simulink model "TwoLinkCartesianNN"  (Simulink 7.6)
settings: Solver=ode45  StartTime=0.0  StopTime=10.0  RelTol=1e-3
libraries: neural x148, roblocks x3, simulink x1
(part 4 of 5)

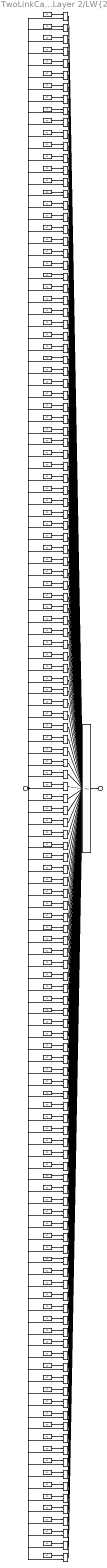
== system TwoLinkCartesianNN/Custom Neural Network/Layer 2/LW{2,1} ==
  "ad{2,1}" : Inport  PortDimensions=10
      mask Display: e = 0.06;c1 = [120 230 180]/255;c2 = ([120 230 180]+0)/(256+128);c3 = ([120 230 180]+128)/(256+128);patch([0 1 1 0],[0 0 1 1],c1);patch([0 1 1 1-e 1-e 0+e],[0 0 1 1-e 0+e 0+e],c2);patch([0 0 1 1-e 0+e 0+e],[0 1 1 1-e 1-e 0+e],c3);plot([0 1 1 0 0],[0 0 1 1 0]);
  "IW{2,1}(1,:)'" : Constant  Value=[1.3771051605919495397500895705888979136943817138671875;1.4379727812980205303716729758889414370059967041015625;-0.71484904480061584042260847127181477844715118408203125;0.195728691276192190429128459072671830654144287109375;-1.40204187084294051857114027370698750019073486328125;-0.0711414545212695481612996672993176616728305816650390625;-0.77472100986854341986287408872158266603946685791015625;1.489410727801894207544819437316618859767913818359375;1.715302916655259135580990914604626595973968505859375;2.718694540405024451246163152973167598247528076171875]
      mask Display: e = 0.06;c1 = [120 150 230]/255;c2 = ([120 150 230]+0)/383;c3 = ([120 150 230]+128)/383;patch([0 1 1 0],[0 0 1 1],c1);patch([0 1 1 1-e 1-e 0+e],[0 0 1 1-e 0+e 0+e],c2);patch([0 0 1 1-e 0+e 0+e],[0 1 1 1-e 1-e 0+e],c3);plot([0 1 1 0 0],[0 0 1 1 0]);disp('weights');
  "IW{2,1}(10,:)'" : Constant  Value=[-1.049488522602133766525867031305097043514251708984375;1.16658805918520958044837243505753576755523681640625;-0.79840961629492712692268696628161706030368804931640625;-0.596367663897474198364534458960406482219696044921875;1.558993573274443544818268492235802114009857177734375;-0.5828639335874774562995526139275170862674713134765625;2.034904616688063327956115244887769222259521484375;-0.74732958615957112424865727007272653281688690185546875;1.8705078039982783177919145600753836333751678466796875;0.39898729108689867661752259664353914558887481689453125]
      mask Display: e = 0.06;c1 = [120 150 230]/255;c2 = ([120 150 230]+0)/383;c3 = ([120 150 230]+128)/383;patch([0 1 1 0],[0 0 1 1],c1);patch([0 1 1 1-e 1-e 0+e],[0 0 1 1-e 0+e 0+e],c2);patch([0 0 1 1-e 0+e 0+e],[0 1 1 1-e 1-e 0+e],c3);plot([0 1 1 0 0],[0 0 1 1 0]);disp('weights');
  "IW{2,1}(100,:)'" : Constant  Value=[-1.225944562580657315464804923976771533489227294921875;0.8399160095312352414254064569831825792789459228515625;0.4059314815768413353680443833582103252410888671875;2.245993199122457983918366153375245630741119384765625;-1.34935754592711010246830483083613216876983642578125;0.88606781850175642123446095865801908075809478759765625;-0.49755438593116918521985780898830853402614593505859375;-2.13120059899219693733130043256096541881561279296875;0.70410764783046941861499590231687761843204498291015625;0.51899870794404001639321677430416457355022430419921875]
      mask Display: e = 0.06;c1 = [120 150 230]/255;c2 = ([120 150 230]+0)/383;c3 = ([120 150 230]+128)/383;patch([0 1 1 0],[0 0 1 1],c1);patch([0 1 1 1-e 1-e 0+e],[0 0 1 1-e 0+e 0+e],c2);patch([0 0 1 1-e 0+e 0+e],[0 1 1 1-e 1-e 0+e],c3);plot([0 1 1 0 0],[0 0 1 1 0]);disp('weights');
  "IW{2,1}(101,:)'" : Constant  Value=[-0.1714405387687350235115246732675586827099323272705078125;-1.843339039992688999092251833644695580005645751953125;0.7673938264733717318222261383198201656341552734375;0.28768398362630309694765173844643868505954742431640625;-1.064859588474557750004123590770177543163299560546875;1.0058133839706095979948941021575592458248138427734375;0.49729546415479652932134513321216218173503875732421875;0.7812040402926265780791936776950024068355560302734375;-1.448282334202080079421648406423628330230712890625;-1.604786002596785277063418106990866363048553466796875]
      mask Display: e = 0.06;c1 = [120 150 230]/255;c2 = ([120 150 230]+0)/383;c3 = ([120 150 230]+128)/383;patch([0 1 1 0],[0 0 1 1],c1);patch([0 1 1 1-e 1-e 0+e],[0 0 1 1-e 0+e 0+e],c2);patch([0 0 1 1-e 0+e 0+e],[0 1 1 1-e 1-e 0+e],c3);plot([0 1 1 0 0],[0 0 1 1 0]);disp('weights');
  "IW{2,1}(102,:)'" : Constant  Value=[-1.2545233242325242173365040798671543598175048828125;-0.894476023393375729853005395852960646152496337890625;1.1069829896758041076765266552683897316455841064453125;0.147037052165285342386624733990174718201160430908203125;-0.9477795368044692470022027919185347855091094970703125;2.607048561729722990776281221769750118255615234375;-0.72985079928825002948400424429564736783504486083984375;0.706545092454415879501539166085422039031982421875;-0.30928314913333299074338356149382889270782470703125;0.3647013350823404831402285708463750779628753662109375]
      mask Display: e = 0.06;c1 = [120 150 230]/255;c2 = ([120 150 230]+0)/383;c3 = ([120 150 230]+128)/383;patch([0 1 1 0],[0 0 1 1],c1);patch([0 1 1 1-e 1-e 0+e],[0 0 1 1-e 0+e 0+e],c2);patch([0 0 1 1-e 0+e 0+e],[0 1 1 1-e 1-e 0+e],c3);plot([0 1 1 0 0],[0 0 1 1 0]);disp('weights');
  "IW{2,1}(103,:)'" : Constant  Value=[-1.94836898360320720513527703587897121906280517578125;-0.99346656875890848592547399675822816789150238037109375;0.6289366685263091394375578602193854749202728271484375;0.296923346045088909495035522922989912331104278564453125;-2.082237542107012728820336633361876010894775390625;0.74701207285368997901287002605386078357696533203125;0.04587202544748684995834508981715771369636058807373046875;0.189311271141696213504701518104411661624908447265625;-0.625343482234573144751266227103769779205322265625;1.856483616450850693269103430793620645999908447265625]
      mask Display: e = 0.06;c1 = [120 150 230]/255;c2 = ([120 150 230]+0)/383;c3 = ([120 150 230]+128)/383;patch([0 1 1 0],[0 0 1 1],c1);patch([0 1 1 1-e 1-e 0+e],[0 0 1 1-e 0+e 0+e],c2);patch([0 0 1 1-e 0+e 0+e],[0 1 1 1-e 1-e 0+e],c3);plot([0 1 1 0 0],[0 0 1 1 0]);disp('weights');
  "IW{2,1}(104,:)'" : Constant  Value=[-0.87456547307661292034453026644769124686717987060546875;0.661425913822359934357564270612783730030059814453125;-0.91627600934355923900653806413174606859683990478515625;1.394861790653333599721008795313537120819091796875;-1.1510944410415040461970193064189516007900238037109375;1.170013503581202929382243382860906422138214111328125;-1.8531144292825152408710209783748723566532135009765625;-0.2259232537701945930930236272615729831159114837646484375;-1.046011759388601358722326040151529014110565185546875;0.6513090719436076536652535651228390634059906005859375]
      mask Display: e = 0.06;c1 = [120 150 230]/255;c2 = ([120 150 230]+0)/383;c3 = ([120 150 230]+128)/383;patch([0 1 1 0],[0 0 1 1],c1);patch([0 1 1 1-e 1-e 0+e],[0 0 1 1-e 0+e 0+e],c2);patch([0 0 1 1-e 0+e 0+e],[0 1 1 1-e 1-e 0+e],c3);plot([0 1 1 0 0],[0 0 1 1 0]);disp('weights');
  "IW{2,1}(105,:)'" : Constant  Value=[-1.094209185208672163724941128748469054698944091796875;0.49548420203191556598909528474905528128147125244140625;-0.032611187696143517644742360062082298099994659423828125;0.1343534135577627852686788401115336455404758453369140625;-2.804578434152290355996228754520416259765625;0.8665819627705080296919959437218494713306427001953125;-1.58400745771962991881309790187515318393707275390625;-1.0376011747574775956337589377653785049915313720703125;0.51815544679734848454444318122114054858684539794921875;0.28060052548613156897516773824463598430156707763671875]
      mask Display: e = 0.06;c1 = [120 150 230]/255;c2 = ([120 150 230]+0)/383;c3 = ([120 150 230]+128)/383;patch([0 1 1 0],[0 0 1 1],c1);patch([0 1 1 1-e 1-e 0+e],[0 0 1 1-e 0+e 0+e],c2);patch([0 0 1 1-e 0+e 0+e],[0 1 1 1-e 1-e 0+e],c3);plot([0 1 1 0 0],[0 0 1 1 0]);disp('weights');
  "IW{2,1}(106,:)'" : Constant  Value=[-1.0412189271557139580437478798558004200458526611328125;-1.3436639474912179803567369162919931113719940185546875;0.450010126140095056967993514263071119785308837890625;0.6522412840593958538448760009487159550189971923828125;-1.3690007423795409469136075131245888769626617431640625;1.7553318938817750183289945198339410126209259033203125;-0.52816214245538783966793516810867004096508026123046875;0.68254375334420636090015932495589368045330047607421875;0.1899048648480208267841362612671218812465667724609375;0.46489516803753005991239888317068107426166534423828125]
      mask Display: e = 0.06;c1 = [120 150 230]/255;c2 = ([120 150 230]+0)/383;c3 = ([120 150 230]+128)/383;patch([0 1 1 0],[0 0 1 1],c1);patch([0 1 1 1-e 1-e 0+e],[0 0 1 1-e 0+e 0+e],c2);patch([0 0 1 1-e 0+e 0+e],[0 1 1 1-e 1-e 0+e],c3);plot([0 1 1 0 0],[0 0 1 1 0]);disp('weights');
  "IW{2,1}(107,:)'" : Constant  Value=[0.153973820406076045141929853343754075467586517333984375;0.59276840590438961697827835450880229473114013671875;0.7783307428557326712592612238950096070766448974609375;0.7722750255361525706376824018661864101886749267578125;-1.1928105881029418267047503832145594060420989990234375;0.99759757590523390202719156150124035775661468505859375;-1.022952057266451220129965804517269134521484375;-1.257958029793900589510258214431814849376678466796875;-1.044800312874491599046677947626449167728424072265625;0.7449342018252840258440983234322629868984222412109375]
      mask Display: e = 0.06;c1 = [120 150 230]/255;c2 = ([120 150 230]+0)/383;c3 = ([120 150 230]+128)/383;patch([0 1 1 0],[0 0 1 1],c1);patch([0 1 1 1-e 1-e 0+e],[0 0 1 1-e 0+e 0+e],c2);patch([0 0 1 1-e 0+e 0+e],[0 1 1 1-e 1-e 0+e],c3);plot([0 1 1 0 0],[0 0 1 1 0]);disp('weights');
  "IW{2,1}(108,:)'" : Constant  Value=[-0.317270268462206406212544607114978134632110595703125;-0.78234381860883084325308800544007681310176849365234375;1.4109189007603524235179293100372888147830963134765625;0.54527910955896119471475458340137265622615814208984375;-1.7025481621260001308115761275985278189182281494140625;-0.0346614276375626084725212194825871847569942474365234375;-1.2100164522013028278735191634041257202625274658203125;-1.6024458763814621864440823628683574497699737548828125;0.177985470391995637129411989008076488971710205078125;0.231119941888123847650859943314571864902973175048828125]
      mask Display: e = 0.06;c1 = [120 150 230]/255;c2 = ([120 150 230]+0)/383;c3 = ([120 150 230]+128)/383;patch([0 1 1 0],[0 0 1 1],c1);patch([0 1 1 1-e 1-e 0+e],[0 0 1 1-e 0+e 0+e],c2);patch([0 0 1 1-e 0+e 0+e],[0 1 1 1-e 1-e 0+e],c3);plot([0 1 1 0 0],[0 0 1 1 0]);disp('weights');
  "IW{2,1}(109,:)'" : Constant  Value=[-0.5582295377645578593472919237683527171611785888671875;-0.94867965993962410919948524679057300090789794921875;2.057364756568237584843927834299392998218536376953125;-0.98615375447739828107529547196463681757450103759765625;-0.7135560563744836048982733700540848076343536376953125;0.766056608937204952525235057692043483257293701171875;0.4477081483988667454099186215898953378200531005859375;0.477742528556733880851226103914086706936359405517578125;-1.774251596140266951096009506727568805217742919921875;-1.2966009978867789609324745470075868070125579833984375]
      mask Display: e = 0.06;c1 = [120 150 230]/255;c2 = ([120 150 230]+0)/383;c3 = ([120 150 230]+128)/383;patch([0 1 1 0],[0 0 1 1],c1);patch([0 1 1 1-e 1-e 0+e],[0 0 1 1-e 0+e 0+e],c2);patch([0 0 1 1-e 0+e 0+e],[0 1 1 1-e 1-e 0+e],c3);plot([0 1 1 0 0],[0 0 1 1 0]);disp('weights');
  "IW{2,1}(11,:)'" : Constant  Value=[0.5708548919310076907862594453035853803157806396484375;0.2994503435388351508805726552964188158512115478515625;0.05453966227569835567567935186161776073276996612548828125;3.535713422952375228902610615477897226810455322265625;-0.9746812457350657599164378552814014256000518798828125;2.701823536859901508933035074733197689056396484375;-1.9659770683795965151574591800454072654247283935546875;-0.40610966247299729037223414707113988697528839111328125;-0.52866074015094233207179286182508803904056549072265625;-0.37017130778386320155703970158356241881847381591796875]
      mask Display: e = 0.06;c1 = [120 150 230]/255;c2 = ([120 150 230]+0)/383;c3 = ([120 150 230]+128)/383;patch([0 1 1 0],[0 0 1 1],c1);patch([0 1 1 1-e 1-e 0+e],[0 0 1 1-e 0+e 0+e],c2);patch([0 0 1 1-e 0+e 0+e],[0 1 1 1-e 1-e 0+e],c3);plot([0 1 1 0 0],[0 0 1 1 0]);disp('weights');
  "IW{2,1}(110,:)'" : Constant  Value=[-0.463559492431017738933718419502838514745235443115234375;-1.286969684233489896740820768172852694988250732421875;-0.7079101718954798894145596932503394782543182373046875;0.307732483292716463285643158087623305618762969970703125;-2.00421019960866697573464989545755088329315185546875;0.925330919989983069484651423408649861812591552734375;0.18853837556779973194664989932789467275142669677734375;-1.3655274693134009655892668888554908335208892822265625;-1.17515447133861616890726509154774248600006103515625;-0.441615151407447503739689409485436044633388519287109375]
      mask Display: e = 0.06;c1 = [120 150 230]/255;c2 = ([120 150 230]+0)/383;c3 = ([120 150 230]+128)/383;patch([0 1 1 0],[0 0 1 1],c1);patch([0 1 1 1-e 1-e 0+e],[0 0 1 1-e 0+e 0+e],c2);patch([0 0 1 1-e 0+e 0+e],[0 1 1 1-e 1-e 0+e],c3);plot([0 1 1 0 0],[0 0 1 1 0]);disp('weights');
  "IW{2,1}(111,:)'" : Constant  Value=[-0.86950100145730047085379510463098995387554168701171875;-0.086003733886987399070989113170071505010128021240234375;1.4885507325407034695530228418647311627864837646484375;-0.160595157190656812051798851825878955423831939697265625;-0.92629070090353626820700583266443572938442230224609375;1.7936429395870086000996934672002680599689483642578125;-0.82718478772733006199047167683602310717105865478515625;-1.49128305220387691321093370788730680942535400390625;-1.4678418857357977689304107116186060011386871337890625;-0.30604727166511980218643884654738940298557281494140625]
      mask Display: e = 0.06;c1 = [120 150 230]/255;c2 = ([120 150 230]+0)/383;c3 = ([120 150 230]+128)/383;patch([0 1 1 0],[0 0 1 1],c1);patch([0 1 1 1-e 1-e 0+e],[0 0 1 1-e 0+e 0+e],c2);patch([0 0 1 1-e 0+e 0+e],[0 1 1 1-e 1-e 0+e],c3);plot([0 1 1 0 0],[0 0 1 1 0]);disp('weights');
  "IW{2,1}(112,:)'" : Constant  Value=[0.08673762663269568573554124668589793145656585693359375;-0.482157669897441520934222580763162113726139068603515625;1.3448576151122064725740301582845859229564666748046875;0.08995801031965877658791441717767156660556793212890625;-0.3390982107780746712677455434459261596202850341796875;-0.1837160523452606997185654336135485209524631500244140625;-0.51843880063664637969367277037235908210277557373046875;0.297759743443221924774633180277305655181407928466796875;-2.26903573696061133802004405879415571689605712890625;-3.179293141307128589545527574955485761165618896484375]
      mask Display: e = 0.06;c1 = [120 150 230]/255;c2 = ([120 150 230]+0)/383;c3 = ([120 150 230]+128)/383;patch([0 1 1 0],[0 0 1 1],c1);patch([0 1 1 1-e 1-e 0+e],[0 0 1 1-e 0+e 0+e],c2);patch([0 0 1 1-e 0+e 0+e],[0 1 1 1-e 1-e 0+e],c3);plot([0 1 1 0 0],[0 0 1 1 0]);disp('weights');
  "IW{2,1}(113,:)'" : Constant  Value=[-0.13866243203950634477195080762612633407115936279296875;-0.903076028083175774696655935258604586124420166015625;0.5088759928895136841475732580875046551227569580078125;-1.3942096726953590035691377124749124050140380859375;-1.47508193731302572615504686837084591388702392578125;1.030490659825020305362386352499015629291534423828125;0.0559448512287377963669854352701804600656032562255859375;-1.2023622777319626919734218972735106945037841796875;-1.7498178193257045709430030910880304872989654541015625;0.11383380590557556910624725787783972918987274169921875]
      mask Display: e = 0.06;c1 = [120 150 230]/255;c2 = ([120 150 230]+0)/383;c3 = ([120 150 230]+128)/383;patch([0 1 1 0],[0 0 1 1],c1);patch([0 1 1 1-e 1-e 0+e],[0 0 1 1-e 0+e 0+e],c2);patch([0 0 1 1-e 0+e 0+e],[0 1 1 1-e 1-e 0+e],c3);plot([0 1 1 0 0],[0 0 1 1 0]);disp('weights');
  "IW{2,1}(114,:)'" : Constant  Value=[-0.68103564413836370494692573629436083137989044189453125;0.2454540755634809501284365751416771672666072845458984375;0.129133428570527619694274790163035504519939422607421875;-0.65105668156396057089096984782372601330280303955078125;-1.384640645282240623004099688841961324214935302734375;2.31729652203841762769798151566646993160247802734375;-1.73033498072638369791320656077004969120025634765625;-0.3600660164124940276764164082123897969722747802734375;-0.214882027578012835267173841202748008072376251220703125;-0.002626066509351120126236622809301479719579219818115234375]
      mask Display: e = 0.06;c1 = [120 150 230]/255;c2 = ([120 150 230]+0)/383;c3 = ([120 150 230]+128)/383;patch([0 1 1 0],[0 0 1 1],c1);patch([0 1 1 1-e 1-e 0+e],[0 0 1 1-e 0+e 0+e],c2);patch([0 0 1 1-e 0+e 0+e],[0 1 1 1-e 1-e 0+e],c3);plot([0 1 1 0 0],[0 0 1 1 0]);disp('weights');
  "IW{2,1}(115,:)'" : Constant  Value=[0.3405733341700345473412880892283283174037933349609375;0.1443005511043800037640494338120333850383758544921875;0.421896751264511704615500775616965256631374359130859375;0.19503977769952551835075382768991403281688690185546875;-1.0749186433771600324149630978354252874851226806640625;1.5814869514372758008136088392348028719425201416015625;-1.519113126773008470848935758112929761409759521484375;0.288997665278035775759946091056917794048786163330078125;-1.405768760662715610720852055237628519535064697265625;-0.452806643977210654394838229563902132213115692138671875]
      mask Display: e = 0.06;c1 = [120 150 230]/255;c2 = ([120 150 230]+0)/383;c3 = ([120 150 230]+128)/383;patch([0 1 1 0],[0 0 1 1],c1);patch([0 1 1 1-e 1-e 0+e],[0 0 1 1-e 0+e 0+e],c2);patch([0 0 1 1-e 0+e 0+e],[0 1 1 1-e 1-e 0+e],c3);plot([0 1 1 0 0],[0 0 1 1 0]);disp('weights');
  "IW{2,1}(116,:)'" : Constant  Value=[0.65285187341882477962684561134665273129940032958984375;-0.9361362991940269662194396005361340939998626708984375;0.30231395696110097137676575584919191896915435791015625;-1.775221877795830405233346027671359479427337646484375;0.474600774354878407468305567817878909409046173095703125;-2.37387731492440412495170676265843212604522705078125;0.9319850982036921305251553349080495536327362060546875;2.76621300569181105544203091994859278202056884765625;0.243678949355843499358087456130306236445903778076171875;0.5861485922523070879464057725272141396999359130859375]
      mask Display: e = 0.06;c1 = [120 150 230]/255;c2 = ([120 150 230]+0)/383;c3 = ([120 150 230]+128)/383;patch([0 1 1 0],[0 0 1 1],c1);patch([0 1 1 1-e 1-e 0+e],[0 0 1 1-e 0+e 0+e],c2);patch([0 0 1 1-e 0+e 0+e],[0 1 1 1-e 1-e 0+e],c3);plot([0 1 1 0 0],[0 0 1 1 0]);disp('weights');
  "IW{2,1}(117,:)'" : Constant  Value=[0.9455838655038875106839668660541065037250518798828125;-0.281727372152586752473979458955000154674053192138671875;0.378485022523104397418336475311662070453166961669921875;0.1781024643238760252206276391007122583687305450439453125;1.963660955691367338005193232675082981586456298828125;-1.955949345100926439755539831821806728839874267578125;0.64078211411344121462008160960976965725421905517578125;1.3135598738807787722038256106316111981868743896484375;0.85956716793419507549600666607148014008998870849609375;-0.35347177839313814740052066554198972880840301513671875]
      mask Display: e = 0.06;c1 = [120 150 230]/255;c2 = ([120 150 230]+0)/383;c3 = ([120 150 230]+128)/383;patch([0 1 1 0],[0 0 1 1],c1);patch([0 1 1 1-e 1-e 0+e],[0 0 1 1-e 0+e 0+e],c2);patch([0 0 1 1-e 0+e 0+e],[0 1 1 1-e 1-e 0+e],c3);plot([0 1 1 0 0],[0 0 1 1 0]);disp('weights');
  "IW{2,1}(118,:)'" : Constant  Value=[0.981526938132869730679885833524167537689208984375;0.1854496983447053437554785659813205711543560028076171875;-1.1169080902003951649703594739548861980438232421875;-1.860445028099551922906584877637214958667755126953125;-0.0460237019197944074999639951784047298133373260498046875;-1.0552251865630417615449232471291907131671905517578125;1.7317393047462059652019661371014080941677093505859375;0.41331953096930529323316250156494788825511932373046875;-0.31436557615315374736297826530062593519687652587890625;-1.1971753010706105424532097458723001182079315185546875]
      mask Display: e = 0.06;c1 = [120 150 230]/255;c2 = ([120 150 230]+0)/383;c3 = ([120 150 230]+128)/383;patch([0 1 1 0],[0 0 1 1],c1);patch([0 1 1 1-e 1-e 0+e],[0 0 1 1-e 0+e 0+e],c2);patch([0 0 1 1-e 0+e 0+e],[0 1 1 1-e 1-e 0+e],c3);plot([0 1 1 0 0],[0 0 1 1 0]);disp('weights');
  "IW{2,1}(119,:)'" : Constant  Value=[0.4649451149538952332562757874256931245326995849609375;1.1253069860781621525092077717999927699565887451171875;0.142656092563263114936233932894538156688213348388671875;-0.228438044279885288379006169634521938860416412353515625;1.2656807856995599959049059179960750043392181396484375;0.0935106467688479880973062563498388044536113739013671875;1.3319995158088406839169692830182611942291259765625;-0.51355059551954607144352848990820348262786865234375;1.7512100372819949800629046876565553247928619384765625;1.7871946660724644662110449644387699663639068603515625]
      mask Display: e = 0.06;c1 = [120 150 230]/255;c2 = ([120 150 230]+0)/383;c3 = ([120 150 230]+128)/383;patch([0 1 1 0],[0 0 1 1],c1);patch([0 1 1 1-e 1-e 0+e],[0 0 1 1-e 0+e 0+e],c2);patch([0 0 1 1-e 0+e 0+e],[0 1 1 1-e 1-e 0+e],c3);plot([0 1 1 0 0],[0 0 1 1 0]);disp('weights');
  "IW{2,1}(12,:)'" : Constant  Value=[0.44903879819862002609198725622263737022876739501953125;0.1351886846011068621375983411780907772481441497802734375;1.42962882355686726754129267646931111812591552734375;0.327571594047642411506870985249406658113002777099609375;-1.4481656703343024350516543563571758568286895751953125;0.421682959239582599852980138166458345949649810791015625;-1.4960126128457693628348579295561648905277252197265625;-0.945237174079860853481704907608218491077423095703125;-0.44385215514368103750797445172793231904506683349609375;-0.010862598242713315810359375745974830351769924163818359375]
      mask Display: e = 0.06;c1 = [120 150 230]/255;c2 = ([120 150 230]+0)/383;c3 = ([120 150 230]+128)/383;patch([0 1 1 0],[0 0 1 1],c1);patch([0 1 1 1-e 1-e 0+e],[0 0 1 1-e 0+e 0+e],c2);patch([0 0 1 1-e 0+e 0+e],[0 1 1 1-e 1-e 0+e],c3);plot([0 1 1 0 0],[0 0 1 1 0]);disp('weights');
  "IW{2,1}(120,:)'" : Constant  Value=[1.1396274870924785194148398659308440983295440673828125;1.0734647864884412360453325163689441978931427001953125;-0.6137086272248357676772911872831173241138458251953125;0.069959460747333779284673482834477908909320831298828125;2.879856829030032816518769323010928928852081298828125;-0.7395936728521521619228451527305878698825836181640625;0.107536844018245592025095902499742805957794189453125;0.85008408760152354144423725301749072968959808349609375;-0.1498745413754074273793293059497955255210399627685546875;-1.1386238501003302925340676665655337274074554443359375]
      mask Display: e = 0.06;c1 = [120 150 230]/255;c2 = ([120 150 230]+0)/383;c3 = ([120 150 230]+128)/383;patch([0 1 1 0],[0 0 1 1],c1);patch([0 1 1 1-e 1-e 0+e],[0 0 1 1-e 0+e 0+e],c2);patch([0 0 1 1-e 0+e 0+e],[0 1 1 1-e 1-e 0+e],c3);plot([0 1 1 0 0],[0 0 1 1 0]);disp('weights');
  "IW{2,1}(121,:)'" : Constant  Value=[0.815964649013100729035841141012497246265411376953125;-0.30130916776370486598324305305141024291515350341796875;0.882263162055509919667883877991698682308197021484375;-2.2345912320881069490496884100139141082763671875;1.928626466044280451939130216487683355808258056640625;-0.97318597578985344132007639927905984222888946533203125;1.4661645219842014409294961296836845576763153076171875;1.1734728362201247708895834875875152647495269775390625;-1.267601876728301935060017058276571333408355712890625;-0.439554158973339437199712165238452143967151641845703125]
      mask Display: e = 0.06;c1 = [120 150 230]/255;c2 = ([120 150 230]+0)/383;c3 = ([120 150 230]+128)/383;patch([0 1 1 0],[0 0 1 1],c1);patch([0 1 1 1-e 1-e 0+e],[0 0 1 1-e 0+e 0+e],c2);patch([0 0 1 1-e 0+e 0+e],[0 1 1 1-e 1-e 0+e],c3);plot([0 1 1 0 0],[0 0 1 1 0]);disp('weights');
  "IW{2,1}(122,:)'" : Constant  Value=[0.74310863823133532779507959276088513433933258056640625;-0.66221907246191447082850345395854674279689788818359375;-1.5289167018819489474168449305579997599124908447265625;0.78506255062807406286395917049958370625972747802734375;2.67636379517875955258432441041804850101470947265625;-0.83146940220393872333914941918919794261455535888671875;1.4270133616463820391828676292789168655872344970703125;-0.61085279523542845847572380080237053334712982177734375;0.996242388806183765126434082048945128917694091796875;-0.97302044175134272396832102458574809134006500244140625]
      mask Display: e = 0.06;c1 = [120 150 230]/255;c2 = ([120 150 230]+0)/383;c3 = ([120 150 230]+128)/383;patch([0 1 1 0],[0 0 1 1],c1);patch([0 1 1 1-e 1-e 0+e],[0 0 1 1-e 0+e 0+e],c2);patch([0 0 1 1-e 0+e 0+e],[0 1 1 1-e 1-e 0+e],c3);plot([0 1 1 0 0],[0 0 1 1 0]);disp('weights');
  "IW{2,1}(123,:)'" : Constant  Value=[-0.249078378358074503662322740638046525418758392333984375;-0.482565969165921149208742235714453272521495819091796875;-1.136723135972611320454461747431196272373199462890625;-0.38062912314735919405705999452038668096065521240234375;1.531287854728446973240352235734462738037109375;-1.1811668496914349280046963031054474413394927978515625;0.001177681898394990211986765871188254095613956451416015625;0.67911567169289799306142185741919092833995819091796875;1.3748533616058062900577851905836723744869232177734375;1.6686272857557014059892708246479742228984832763671875]
      mask Display: e = 0.06;c1 = [120 150 230]/255;c2 = ([120 150 230]+0)/383;c3 = ([120 150 230]+128)/383;patch([0 1 1 0],[0 0 1 1],c1);patch([0 1 1 1-e 1-e 0+e],[0 0 1 1-e 0+e 0+e],c2);patch([0 0 1 1-e 0+e 0+e],[0 1 1 1-e 1-e 0+e],c3);plot([0 1 1 0 0],[0 0 1 1 0]);disp('weights');
  "IW{2,1}(124,:)'" : Constant  Value=[0.1401144544971815175671281394897960126399993896484375;0.66890064779860247679010853971703909337520599365234375;-1.948365491313690522900969881447963416576385498046875;-0.45989159942316859552846608494292013347148895263671875;1.398363758177370907986869497108273208141326904296875;-0.53727942193003297433051557163707911968231201171875;0.86314530188005156308150844779447652399539947509765625;1.6426498249198804302295684465207159519195556640625;1.1051033795981977103650706339976750314235687255859375;-0.1103368485235165230573528560853446833789348602294921875]
      mask Display: e = 0.06;c1 = [120 150 230]/255;c2 = ([120 150 230]+0)/383;c3 = ([120 150 230]+128)/383;patch([0 1 1 0],[0 0 1 1],c1);patch([0 1 1 1-e 1-e 0+e],[0 0 1 1-e 0+e 0+e],c2);patch([0 0 1 1-e 0+e 0+e],[0 1 1 1-e 1-e 0+e],c3);plot([0 1 1 0 0],[0 0 1 1 0]);disp('weights');
  "IW{2,1}(125,:)'" : Constant  Value=[2.037858645567606430404339334927499294281005859375;-0.92816942111053057917757769246236421167850494384765625;-1.2295234454379742050633694816497154533863067626953125;-1.662571349093350026038251598947681486606597900390625;2.787946025089679036312872995040379464626312255859375;-2.223514561837401704025296567124314606189727783203125;1.2518297971880991692472662180080078542232513427734375;1.0325664823558617921861468857969157397747039794921875;3.0022481067670714338646575924940407276153564453125;2.754995413226974942944025315227918326854705810546875]
      mask Display: e = 0.06;c1 = [120 150 230]/255;c2 = ([120 150 230]+0)/383;c3 = ([120 150 230]+128)/383;patch([0 1 1 0],[0 0 1 1],c1);patch([0 1 1 1-e 1-e 0+e],[0 0 1 1-e 0+e 0+e],c2);patch([0 0 1 1-e 0+e 0+e],[0 1 1 1-e 1-e 0+e],c3);plot([0 1 1 0 0],[0 0 1 1 0]);disp('weights');
  "IW{2,1}(126,:)'" : Constant  Value=[1.2556150090851769807187565675121732056140899658203125;-0.507004608863867556323157259612344205379486083984375;0.0225493146456884618888949489701190032064914703369140625;-2.39119867429262722424709863844327628612518310546875;2.841519818610972691885763197205960750579833984375;-1.129013556368041459876394583261571824550628662109375;0.0450215685549583966018616365545312874019145965576171875;1.1222970193774497449368254820001311600208282470703125;-0.89280273915049035426960699624032713472843170166015625;-0.266809595345054384463168162255897186696529388427734375]
      mask Display: e = 0.06;c1 = [120 150 230]/255;c2 = ([120 150 230]+0)/383;c3 = ([120 150 230]+128)/383;patch([0 1 1 0],[0 0 1 1],c1);patch([0 1 1 1-e 1-e 0+e],[0 0 1 1-e 0+e 0+e],c2);patch([0 0 1 1-e 0+e 0+e],[0 1 1 1-e 1-e 0+e],c3);plot([0 1 1 0 0],[0 0 1 1 0]);disp('weights');
  "IW{2,1}(127,:)'" : Constant  Value=[-0.280124086206472278082202365112607367336750030517578125;1.077790205652555233228895303909666836261749267578125;-1.0949528423733625448477368991007097065448760986328125;0.501459573955923332277961890213191509246826171875;3.462127080873177664699369415757246315479278564453125;-2.546824016381276312159798180800862610340118408203125;0.0801562068816956407868445921849342994391918182373046875;2.661437784930992922483028451097197830677032470703125;0.05809000935187276504212405825455789454281330108642578125;-4.48477332434274700290188775397837162017822265625]
      mask Display: e = 0.06;c1 = [120 150 230]/255;c2 = ([120 150 230]+0)/383;c3 = ([120 150 230]+128)/383;patch([0 1 1 0],[0 0 1 1],c1);patch([0 1 1 1-e 1-e 0+e],[0 0 1 1-e 0+e 0+e],c2);patch([0 0 1 1-e 0+e 0+e],[0 1 1 1-e 1-e 0+e],c3);plot([0 1 1 0 0],[0 0 1 1 0]);disp('weights');
  "IW{2,1}(128,:)'" : Constant  Value=[1.1415905739136220642393482194165699183940887451171875;-0.1233348779983350074207493207723018713295459747314453125;-1.842810765070568290724395410506986081600189208984375;0.24269383618367446064922887671855278313159942626953125;0.9546868802602823667058373757754452526569366455078125;0.5042679130550322685877517869812436401844024658203125;1.6900310094398065530185704119503498077392578125;0.7042927604097617422240773521480150520801544189453125;1.0990504330900581209107258473522961139678955078125;1.88280021684015874683382207877002656459808349609375]
      mask Display: e = 0.06;c1 = [120 150 230]/255;c2 = ([120 150 230]+0)/383;c3 = ([120 150 230]+128)/383;patch([0 1 1 0],[0 0 1 1],c1);patch([0 1 1 1-e 1-e 0+e],[0 0 1 1-e 0+e 0+e],c2);patch([0 0 1 1-e 0+e 0+e],[0 1 1 1-e 1-e 0+e],c3);plot([0 1 1 0 0],[0 0 1 1 0]);disp('weights');
  "IW{2,1}(129,:)'" : Constant  Value=[0.62596352703475000023303209673031233251094818115234375;-0.4607801523770456153528130016638897359371185302734375;-1.2071285642728895037834035974810831248760223388671875;-0.07087171344364333325227534032819676212966442108154296875;1.802626725986929301370764733292162418365478515625;-1.5761054322224747892278173821978271007537841796875;0.78887816446144498616632745324750430881977081298828125;-0.263377211712159942091915354467346332967281341552734375;1.2227115261267729184879726744838990271091461181640625;0.324718223372467862386514525496750138700008392333984375]
      mask Display: e = 0.06;c1 = [120 150 230]/255;c2 = ([120 150 230]+0)/383;c3 = ([120 150 230]+128)/383;patch([0 1 1 0],[0 0 1 1],c1);patch([0 1 1 1-e 1-e 0+e],[0 0 1 1-e 0+e 0+e],c2);patch([0 0 1 1-e 0+e 0+e],[0 1 1 1-e 1-e 0+e],c3);plot([0 1 1 0 0],[0 0 1 1 0]);disp('weights');
  "IW{2,1}(13,:)'" : Constant  Value=[1.2926177992848246756096841636463068425655364990234375;1.222925930285702289523896979517303407192230224609375;0.02674014673192072477636571647963137365877628326416015625;-1.26652044981072009477429674006998538970947265625;0.51879373893684121998859382074442692101001739501953125;-0.35051318881074566835565065048285759985446929931640625;-0.405709053167195687894519551264238543808460235595703125;1.211619110321688452813759795390069484710693359375;1.1525266439348877955950456453138031065464019775390625;0.695336383375274369456064960104413330554962158203125]
      mask Display: e = 0.06;c1 = [120 150 230]/255;c2 = ([120 150 230]+0)/383;c3 = ([120 150 230]+128)/383;patch([0 1 1 0],[0 0 1 1],c1);patch([0 1 1 1-e 1-e 0+e],[0 0 1 1-e 0+e 0+e],c2);patch([0 0 1 1-e 0+e 0+e],[0 1 1 1-e 1-e 0+e],c3);plot([0 1 1 0 0],[0 0 1 1 0]);disp('weights');
  "IW{2,1}(130,:)'" : Constant  Value=[0.61114815694704949233795332474983297288417816162109375;0.7469798578890414209041637150221504271030426025390625;-0.38742006676732432257637128714122809469699859619140625;-1.8163906077087077495235689639230258762836456298828125;0.211344393439648670085517778716166503727436065673828125;-1.4892539516572380620118565275333821773529052734375;1.170625381969820022476369558717124164104461669921875;0.07442196991290812857489100906605017371475696563720703125;-0.446881337073997020326032725279219448566436767578125;-0.036649961408830707132455728469722089357674121856689453125]
      mask Display: e = 0.06;c1 = [120 150 230]/255;c2 = ([120 150 230]+0)/383;c3 = ([120 150 230]+128)/383;patch([0 1 1 0],[0 0 1 1],c1);patch([0 1 1 1-e 1-e 0+e],[0 0 1 1-e 0+e 0+e],c2);patch([0 0 1 1-e 0+e 0+e],[0 1 1 1-e 1-e 0+e],c3);plot([0 1 1 0 0],[0 0 1 1 0]);disp('weights');
  "IW{2,1}(131,:)'" : Constant  Value=[0.497325299493528272254394551055156625807285308837890625;1.28950718091573524048953913734294474124908447265625;0.0366196892127551854034805955961928702890872955322265625;-2.0284844255546179425664377049542963504791259765625;1.938777328491612994554316173889674246311187744140625;-0.8204173709922633062063823672360740602016448974609375;1.9408241658527629613928411345114000141620635986328125;0.7788995379434011656627490083337761461734771728515625;-0.8358167171329988764938434542273171246051788330078125;-1.002239120940657368663551096688024699687957763671875]
      mask Display: e = 0.06;c1 = [120 150 230]/255;c2 = ([120 150 230]+0)/383;c3 = ([120 150 230]+128)/383;patch([0 1 1 0],[0 0 1 1],c1);patch([0 1 1 1-e 1-e 0+e],[0 0 1 1-e 0+e 0+e],c2);patch([0 0 1 1-e 0+e 0+e],[0 1 1 1-e 1-e 0+e],c3);plot([0 1 1 0 0],[0 0 1 1 0]);disp('weights');
  "IW{2,1}(14,:)'" : Constant  Value=[1.6283212656038552612614012105041183531284332275390625;0.98986635398744449165775449728243984282016754150390625;0.49367000492251478238614481597323901951313018798828125;-3.9264098207753885816373440320603549480438232421875;2.616358287030636109449233117629773914813995361328125;-2.96931154901729232875595698715187609195709228515625;3.7059525190690099094581455574370920658111572265625;3.564018449074596528447500531910918653011322021484375;2.0881580981608696134799174615181982517242431640625;4.47646907903904978098807987407781183719635009765625]
      mask Display: e = 0.06;c1 = [120 150 230]/255;c2 = ([120 150 230]+0)/383;c3 = ([120 150 230]+128)/383;patch([0 1 1 0],[0 0 1 1],c1);patch([0 1 1 1-e 1-e 0+e],[0 0 1 1-e 0+e 0+e],c2);patch([0 0 1 1-e 0+e 0+e],[0 1 1 1-e 1-e 0+e],c3);plot([0 1 1 0 0],[0 0 1 1 0]);disp('weights');
  "IW{2,1}(15,:)'" : Constant  Value=[-0.194545959776940780017184806638397276401519775390625;1.341064920783419989191997956368140876293182373046875;-0.30516363896508391650996827593189664185047149658203125;-1.607298827836300514348977230838499963283538818359375;0.319693149038203727752005534057389013469219207763671875;-1.475595221756897057474589018966071307659149169921875;0.53749075762494025187976376400911249220371246337890625;0.423162565413680746839730772990151308476924896240234375;-0.63229239862675623573551320077967830002307891845703125;1.23222828596601718942338266060687601566314697265625]
      mask Display: e = 0.06;c1 = [120 150 230]/255;c2 = ([120 150 230]+0)/383;c3 = ([120 150 230]+128)/383;patch([0 1 1 0],[0 0 1 1],c1);patch([0 1 1 1-e 1-e 0+e],[0 0 1 1-e 0+e 0+e],c2);patch([0 0 1 1-e 0+e 0+e],[0 1 1 1-e 1-e 0+e],c3);plot([0 1 1 0 0],[0 0 1 1 0]);disp('weights');
  "IW{2,1}(16,:)'" : Constant  Value=[2.042860403032298766134999823407270014286041259765625;0.170559441905617836798825237565324641764163970947265625;-1.27610140749427802830950895440764725208282470703125;-0.00426310843723119725634518317747279070317745208740234375;0.69083914916547417561787369777448475360870361328125;0.75576869628878429185903087272890843451023101806640625;0.197096504188498278242747119293198920786380767822265625;-0.84636373670561948490131953803938813507556915283203125;1.90105605558995538473254782729782164096832275390625;1.619547731009394642143206510809250175952911376953125]
      mask Display: e = 0.06;c1 = [120 150 230]/255;c2 = ([120 150 230]+0)/383;c3 = ([120 150 230]+128)/383;patch([0 1 1 0],[0 0 1 1],c1);patch([0 1 1 1-e 1-e 0+e],[0 0 1 1-e 0+e 0+e],c2);patch([0 0 1 1-e 0+e 0+e],[0 1 1 1-e 1-e 0+e],c3);plot([0 1 1 0 0],[0 0 1 1 0]);disp('weights');
  "IW{2,1}(17,:)'" : Constant  Value=[0.1781724808041762475596669901278801262378692626953125;0.903517550659008517044412656105123460292816162109375;0.1652373656695294290575048989921924658119678497314453125;-2.525991456979199245580502974917180836200714111328125;0.045937331549756273141316142982759629376232624053955078125;-1.921922399383102941783363348804414272308349609375;0.245377947009535357647536102376761846244335174560546875;1.099524154700579625654199844575487077236175537109375;-0.484047241384735371649838953089783899486064910888671875;0.4752729510089903630642993448418565094470977783203125]
      mask Display: e = 0.06;c1 = [120 150 230]/255;c2 = ([120 150 230]+0)/383;c3 = ([120 150 230]+128)/383;patch([0 1 1 0],[0 0 1 1],c1);patch([0 1 1 1-e 1-e 0+e],[0 0 1 1-e 0+e 0+e],c2);patch([0 0 1 1-e 0+e 0+e],[0 1 1 1-e 1-e 0+e],c3);plot([0 1 1 0 0],[0 0 1 1 0]);disp('weights');
  "IW{2,1}(18,:)'" : Constant  Value=[3.4929485768921768595873800222761929035186767578125;1.70912494540989445823697678861208260059356689453125;0.53720482564004534697943427090649493038654327392578125;-0.50434106540715040178923800340271554887294769287109375;1.378614535611891955824148681131191551685333251953125;-2.195641471693793977948416795697994530200958251953125;2.682604936682761120891882455907762050628662109375;1.9780534284378266107751187519170343875885009765625;0.72919348448383802807626352660008706152439117431640625;-2.472022492272277105485045467503368854522705078125]
      mask Display: e = 0.06;c1 = [120 150 230]/255;c2 = ([120 150 230]+0)/383;c3 = ([120 150 230]+128)/383;patch([0 1 1 0],[0 0 1 1],c1);patch([0 1 1 1-e 1-e 0+e],[0 0 1 1-e 0+e 0+e],c2);patch([0 0 1 1-e 0+e 0+e],[0 1 1 1-e 1-e 0+e],c3);plot([0 1 1 0 0],[0 0 1 1 0]);disp('weights');
  "IW{2,1}(19,:)'" : Constant  Value=[0.95375011322692160309344444613088853657245635986328125;0.134794059891906903292380093262181617319583892822265625;-0.51231557359754187341849274162086658179759979248046875;0.7822337748353345165952532624942250549793243408203125;1.6328299183504670910593858934589661657810211181640625;0.0259800375304572173096318010721006430685520172119140625;0.0973316576634468411111100749621982686221599578857421875;1.5940239049697166873187370583764277398586273193359375;1.600023315159828651843554325751028954982757568359375;0.295681148578155805761724650437827222049236297607421875]
      mask Display: e = 0.06;c1 = [120 150 230]/255;c2 = ([120 150 230]+0)/383;c3 = ([120 150 230]+128)/383;patch([0 1 1 0],[0 0 1 1],c1);patch([0 1 1 1-e 1-e 0+e],[0 0 1 1-e 0+e 0+e],c2);patch([0 0 1 1-e 0+e 0+e],[0 1 1 1-e 1-e 0+e],c3);plot([0 1 1 0 0],[0 0 1 1 0]);disp('weights');
  "IW{2,1}(2,:)'" : Constant  Value=[2.067957671620557658087591335061006247997283935546875;-1.5301594590984806121269912182469852268695831298828125;-0.4113842901175857047491035700659267604351043701171875;-1.3096806687040667416255246280343271791934967041015625;3.326728834275452850732790466281585395336151123046875;-0.9879564500103590329871394715155474841594696044921875;0.12922332980014672454416313485126011073589324951171875;0.6259679380700513551261110478662885725498199462890625;1.31953914740563593710476197884418070316314697265625;0.23966544411404366865525616958620958030223846435546875]
      mask Display: e = 0.06;c1 = [120 150 230]/255;c2 = ([120 150 230]+0)/383;c3 = ([120 150 230]+128)/383;patch([0 1 1 0],[0 0 1 1],c1);patch([0 1 1 1-e 1-e 0+e],[0 0 1 1-e 0+e 0+e],c2);patch([0 0 1 1-e 0+e 0+e],[0 1 1 1-e 1-e 0+e],c3);plot([0 1 1 0 0],[0 0 1 1 0]);disp('weights');
  "IW{2,1}(20,:)'" : Constant  Value=[2.088224191248281957911103745573200285434722900390625;-0.050910504055185212823886331534595228731632232666015625;-1.9223994805973323440895228486624546349048614501953125;-0.057892471978255873044094670376580324955284595489501953125;0.99869660984671437820026085319113917648792266845703125;-0.32234596328993081471026016515679657459259033203125;-1.065746336529589388675276495632715523242950439453125;0.1784771429672211973116446870335494168102741241455078125;1.382250985925049580060886000865139067173004150390625;0.8444321740506370854717488327878527343273162841796875]
      mask Display: e = 0.06;c1 = [120 150 230]/255;c2 = ([120 150 230]+0)/383;c3 = ([120 150 230]+128)/383;patch([0 1 1 0],[0 0 1 1],c1);patch([0 1 1 1-e 1-e 0+e],[0 0 1 1-e 0+e 0+e],c2);patch([0 0 1 1-e 0+e 0+e],[0 1 1 1-e 1-e 0+e],c3);plot([0 1 1 0 0],[0 0 1 1 0]);disp('weights');
  "IW{2,1}(21,:)'" : Constant  Value=[0.79673253836783575199120832621701993048191070556640625;1.17183634593089625042239276808686554431915283203125;-2.17736092521773283436914425692521035671234130859375;-0.06057242620870985361225535825724364258348941802978515625;-0.269437582226250083028418202957254834473133087158203125;-0.14657980869759346109759690079954452812671661376953125;-0.34517763588858241252665948195499368011951446533203125;-0.44241496509966016237314079262432642281055450439453125;1.62195588884727204259661448304541409015655517578125;0.6544687251866292410085179653833620250225067138671875]
      mask Display: e = 0.06;c1 = [120 150 230]/255;c2 = ([120 150 230]+0)/383;c3 = ([120 150 230]+128)/383;patch([0 1 1 0],[0 0 1 1],c1);patch([0 1 1 1-e 1-e 0+e],[0 0 1 1-e 0+e 0+e],c2);patch([0 0 1 1-e 0+e 0+e],[0 1 1 1-e 1-e 0+e],c3);plot([0 1 1 0 0],[0 0 1 1 0]);disp('weights');
  "IW{2,1}(22,:)'" : Constant  Value=[1.054885074164368052862528202240355312824249267578125;0.01866265491646533491998383169629960320889949798583984375;0.17883337682902722409750140286632813513278961181640625;-1.157521978738999646196816684096120297908782958984375;-0.21469649659957068532634139046422205865383148193359375;-0.6456731897274206044556876804563216865062713623046875;1.05860087509903788571818950003944337368011474609375;-0.71744577931639852419465341881732456386089324951171875;2.09441883227424074931377617758698761463165283203125;1.347541649090393978127622176543809473514556884765625]
      mask Display: e = 0.06;c1 = [120 150 230]/255;c2 = ([120 150 230]+0)/383;c3 = ([120 150 230]+128)/383;patch([0 1 1 0],[0 0 1 1],c1);patch([0 1 1 1-e 1-e 0+e],[0 0 1 1-e 0+e 0+e],c2);patch([0 0 1 1-e 0+e 0+e],[0 1 1 1-e 1-e 0+e],c3);plot([0 1 1 0 0],[0 0 1 1 0]);disp('weights');
  "IW{2,1}(23,:)'" : Constant  Value=[1.1430799727021503375823385795229114592075347900390625;-0.8351625861337133027717527511413209140300750732421875;-0.00954495967026304514835288728136220015585422515869140625;-1.00143755727593219972959559527225792407989501953125;-0.227964057995669155953777362810797058045864105224609375;-0.40210243529868139322758224807330407202243804931640625;1.804505549491381533044886964489705860614776611328125;1.966571924078383215572785047697834670543670654296875;-0.0589402928616092613989252413375652395188808441162109375;0.599197791961147974149071160354651510715484619140625]
      mask Display: e = 0.06;c1 = [120 150 230]/255;c2 = ([120 150 230]+0)/383;c3 = ([120 150 230]+128)/383;patch([0 1 1 0],[0 0 1 1],c1);patch([0 1 1 1-e 1-e 0+e],[0 0 1 1-e 0+e 0+e],c2);patch([0 0 1 1-e 0+e 0+e],[0 1 1 1-e 1-e 0+e],c3);plot([0 1 1 0 0],[0 0 1 1 0]);disp('weights');
  "IW{2,1}(24,:)'" : Constant  Value=[1.43229008931098800161407780251465737819671630859375;-0.152617536075901949477184871284407563507556915283203125;-1.3545884296600139151678376947529613971710205078125;0.57722994905181790326054169781855307519435882568359375;-0.18385382780908432476252301057684235274791717529296875;0.2784987269016345745598073335713706910610198974609375;1.6467816277569351512966022710315883159637451171875;0.3766039309550446301244619462522678077220916748046875;1.0970002284919420088016295267152599990367889404296875;0.20208152618350727625085028194007463753223419189453125]
      mask Display: e = 0.06;c1 = [120 150 230]/255;c2 = ([120 150 230]+0)/383;c3 = ([120 150 230]+128)/383;patch([0 1 1 0],[0 0 1 1],c1);patch([0 1 1 1-e 1-e 0+e],[0 0 1 1-e 0+e 0+e],c2);patch([0 0 1 1-e 0+e 0+e],[0 1 1 1-e 1-e 0+e],c3);plot([0 1 1 0 0],[0 0 1 1 0]);disp('weights');
  "IW{2,1}(25,:)'" : Constant  Value=[1.4132125080108177694881987918051891028881072998046875;0.8581586846362105891472538132802583277225494384765625;-0.36215556630559309070349627290852367877960205078125;-0.492387803974343951640690875137806870043277740478515625;0.01444692002191250157494550876435823738574981689453125;0.1810819369720307048243768122119945473968982696533203125;1.506065434318544671299378023832105100154876708984375;-0.9183163198152992645617587186279706656932830810546875;1.5114291097917831319108472598600201308727264404296875;1.2809857279270662200332253632950596511363983154296875]
      mask Display: e = 0.06;c1 = [120 150 230]/255;c2 = ([120 150 230]+0)/383;c3 = ([120 150 230]+128)/383;patch([0 1 1 0],[0 0 1 1],c1);patch([0 1 1 1-e 1-e 0+e],[0 0 1 1-e 0+e 0+e],c2);patch([0 0 1 1-e 0+e 0+e],[0 1 1 1-e 1-e 0+e],c3);plot([0 1 1 0 0],[0 0 1 1 0]);disp('weights');
  "IW{2,1}(26,:)'" : Constant  Value=[-0.22619260919548500599063345362083055078983306884765625;0.12422809225192611715105073244558298029005527496337890625;-0.50268793561107727452252902367035858333110809326171875;1.42423155710813009733328726724721491336822509765625;1.8154006400928626163704393547959625720977783203125;-0.513703119476999869874589421669952571392059326171875;2.53896077995674485094923511496745049953460693359375;0.28882948897182114667003816066426225006580352783203125;1.53045848399287276464519891305826604366302490234375;-0.6082758492665174543390094186179339885711669921875]
      mask Display: e = 0.06;c1 = [120 150 230]/255;c2 = ([120 150 230]+0)/383;c3 = ([120 150 230]+128)/383;patch([0 1 1 0],[0 0 1 1],c1);patch([0 1 1 1-e 1-e 0+e],[0 0 1 1-e 0+e 0+e],c2);patch([0 0 1 1-e 0+e 0+e],[0 1 1 1-e 1-e 0+e],c3);plot([0 1 1 0 0],[0 0 1 1 0]);disp('weights');
  "IW{2,1}(27,:)'" : Constant  Value=[-0.6234630377301166870296356137259863317012786865234375;-0.30043843091690269897497955753351561725139617919921875;-1.031084129609787236603324345196597278118133544921875;-1.3906518920918475856751683750189840793609619140625;1.0883457588703908669458542135544121265411376953125;-1.519358489815748836093689533299766480922698974609375;1.5942606356049291438381487751030363142490386962890625;0.482239294244171279313349032236146740615367889404296875;-0.7590998899033183366924504298367537558078765869140625;0.097085303989483395792348119357484392821788787841796875]
      mask Display: e = 0.06;c1 = [120 150 230]/255;c2 = ([120 150 230]+0)/383;c3 = ([120 150 230]+128)/383;patch([0 1 1 0],[0 0 1 1],c1);patch([0 1 1 1-e 1-e 0+e],[0 0 1 1-e 0+e 0+e],c2);patch([0 0 1 1-e 0+e 0+e],[0 1 1 1-e 1-e 0+e],c3);plot([0 1 1 0 0],[0 0 1 1 0]);disp('weights');
  "IW{2,1}(28,:)'" : Constant  Value=[-0.432758377177500597188242181800887919962406158447265625;1.0059378649103278835497121690423227846622467041015625;-1.1943034248217465620456323449616320431232452392578125;-1.6018826030225825629571545505314134061336517333984375;0.810997505598943124738298138254322111606597900390625;-0.6649757685693640230084611175698228180408477783203125;1.491787093894858085008081616251729428768157958984375;0.01246209496918203318838180848615593276917934417724609375;0.206090677443823311332238290560781024396419525146484375;-1.0300454018237361619725334094255231320858001708984375]
      mask Display: e = 0.06;c1 = [120 150 230]/255;c2 = ([120 150 230]+0)/383;c3 = ([120 150 230]+128)/383;patch([0 1 1 0],[0 0 1 1],c1);patch([0 1 1 1-e 1-e 0+e],[0 0 1 1-e 0+e 0+e],c2);patch([0 0 1 1-e 0+e 0+e],[0 1 1 1-e 1-e 0+e],c3);plot([0 1 1 0 0],[0 0 1 1 0]);disp('weights');
  "IW{2,1}(29,:)'" : Constant  Value=[1.6989304862697356401923798330244608223438262939453125;1.385399246641339399133130427799187600612640380859375;0.1179012687544213344725818615188472904264926910400390625;0.4238235050028824613121969377971254289150238037109375;0.9005097841721061424635763614787720143795013427734375;-1.7963667269385055202945977725903503596782684326171875;0.5546060123482161596797368474653922021389007568359375;1.5685599488765313846982962786569260060787200927734375;-0.424581693395234494037282502176822163164615631103515625;0.2105123697913262592606997714028693735599517822265625]
      mask Display: e = 0.06;c1 = [120 150 230]/255;c2 = ([120 150 230]+0)/383;c3 = ([120 150 230]+128)/383;patch([0 1 1 0],[0 0 1 1],c1);patch([0 1 1 1-e 1-e 0+e],[0 0 1 1-e 0+e 0+e],c2);patch([0 0 1 1-e 0+e 0+e],[0 1 1 1-e 1-e 0+e],c3);plot([0 1 1 0 0],[0 0 1 1 0]);disp('weights');
  "IW{2,1}(3,:)'" : Constant  Value=[-0.035806641116365611754446263148565776646137237548828125;-0.0771664067347537507846055859772604890167713165283203125;-1.7441048832377454846920272757415659725666046142578125;-0.29980285046755639211113475539605133235454559326171875;2.886109338503448196178169382619671523571014404296875;-1.675699658951348869351249959436245262622833251953125;1.2832668752688591862209932514815591275691986083984375;1.2411785376354449450531092224991880357265472412109375;0.5768409513768137930611601404962129890918731689453125;-0.8920975405802213931139021951821632683277130126953125]
      mask Display: e = 0.06;c1 = [120 150 230]/255;c2 = ([120 150 230]+0)/383;c3 = ([120 150 230]+128)/383;patch([0 1 1 0],[0 0 1 1],c1);patch([0 1 1 1-e 1-e 0+e],[0 0 1 1-e 0+e 0+e],c2);patch([0 0 1 1-e 0+e 0+e],[0 1 1 1-e 1-e 0+e],c3);plot([0 1 1 0 0],[0 0 1 1 0]);disp('weights');
  "IW{2,1}(30,:)'" : Constant  Value=[-0.03053972651063786847291936510373488999903202056884765625;1.2569955003993051878552478228812105953693389892578125;-1.7286822254871612170035177769022993743419647216796875;1.3650850132751852772372558320057578384876251220703125;0.97182958720843981570425285099190659821033477783203125;-1.1006077949679033967100849622511304914951324462890625;1.0028406150854127787397374049760401248931884765625;0.5384167625553930580650785486795939505100250244140625;0.23184959525451509509963443633751012384891510009765625;-1.03104020320869071980496300966478884220123291015625]
      mask Display: e = 0.06;c1 = [120 150 230]/255;c2 = ([120 150 230]+0)/383;c3 = ([120 150 230]+128)/383;patch([0 1 1 0],[0 0 1 1],c1);patch([0 1 1 1-e 1-e 0+e],[0 0 1 1-e 0+e 0+e],c2);patch([0 0 1 1-e 0+e 0+e],[0 1 1 1-e 1-e 0+e],c3);plot([0 1 1 0 0],[0 0 1 1 0]);disp('weights');
  "IW{2,1}(31,:)'" : Constant  Value=[2.258359285473499955543275063973851501941680908203125;0.25374061647645207440149306421517394483089447021484375;-0.32985100147279222682072941097430884838104248046875;0.75180154680176969339555625992943532764911651611328125;2.307101421729978785180037448299117386341094970703125;-0.465074594170635291501270103253773413598537445068359375;-0.644032529423314681338297305046580731868743896484375;0.466855006872437805487408013505046255886554718017578125;0.640878849807383854653153321123681962490081787109375;1.6785068114789805093778340960852801799774169921875]
      mask Display: e = 0.06;c1 = [120 150 230]/255;c2 = ([120 150 230]+0)/383;c3 = ([120 150 230]+128)/383;patch([0 1 1 0],[0 0 1 1],c1);patch([0 1 1 1-e 1-e 0+e],[0 0 1 1-e 0+e 0+e],c2);patch([0 0 1 1-e 0+e 0+e],[0 1 1 1-e 1-e 0+e],c3);plot([0 1 1 0 0],[0 0 1 1 0]);disp('weights');
  "IW{2,1}(32,:)'" : Constant  Value=[1.2997210079454817321931159312953241169452667236328125;0.64632823076564938080679212362156249582767486572265625;0.63732507418686645817018643356277607381343841552734375;-0.98627072110262792303814194383448921144008636474609375;0.26759553280299430699784579701372422277927398681640625;-0.78815627458760995072140076445066370069980621337890625;0.39757331922941874235988279906450770795345306396484375;0.259259027127001162593700200886814855039119720458984375;1.0181018297362631752633888027048669755458831787109375;2.580754283205482835228394833393394947052001953125]
      mask Display: e = 0.06;c1 = [120 150 230]/255;c2 = ([120 150 230]+0)/383;c3 = ([120 150 230]+128)/383;patch([0 1 1 0],[0 0 1 1],c1);patch([0 1 1 1-e 1-e 0+e],[0 0 1 1-e 0+e 0+e],c2);patch([0 0 1 1-e 0+e 0+e],[0 1 1 1-e 1-e 0+e],c3);plot([0 1 1 0 0],[0 0 1 1 0]);disp('weights');
  "IW{2,1}(33,:)'" : Constant  Value=[-0.686959909739234486636405563331209123134613037109375;0.396707927444221841728477784272399730980396270751953125;-1.6211813519857345422536809564917348325252532958984375;-0.09382042121345603169491056405604467727243900299072265625;1.61389547885149386985403907601721584796905517578125;0.0870282971541260774728243632125668227672576904296875;1.4940966604904974968093256393331103026866912841796875;-0.34571145414237935966639270191080868244171142578125;0.4092217888554883220564306611777283251285552978515625;0.7045828880297990703951427349238656461238861083984375]
      mask Display: e = 0.06;c1 = [120 150 230]/255;c2 = ([120 150 230]+0)/383;c3 = ([120 150 230]+128)/383;patch([0 1 1 0],[0 0 1 1],c1);patch([0 1 1 1-e 1-e 0+e],[0 0 1 1-e 0+e 0+e],c2);patch([0 0 1 1-e 0+e 0+e],[0 1 1 1-e 1-e 0+e],c3);plot([0 1 1 0 0],[0 0 1 1 0]);disp('weights');
  "IW{2,1}(34,:)'" : Constant  Value=[1.1752987742539533488894676338532008230686187744140625;0.47200922024703839685599859876674599945545196533203125;-0.69219136852888019095786376055912114679813385009765625;-0.8767917795579709405728863202966749668121337890625;0.8478135297600111197624528358574025332927703857421875;-0.6561123937294388586138893515453673899173736572265625;-0.12980230239168488726164696345222182571887969970703125;-0.7133411448292441559004828377510420978069305419921875;1.23374113558991016503796345205046236515045166015625;1.633103403422843324932500763679854571819305419921875]
      mask Display: e = 0.06;c1 = [120 150 230]/255;c2 = ([120 150 230]+0)/383;c3 = ([120 150 230]+128)/383;patch([0 1 1 0],[0 0 1 1],c1);patch([0 1 1 1-e 1-e 0+e],[0 0 1 1-e 0+e 0+e],c2);patch([0 0 1 1-e 0+e 0+e],[0 1 1 1-e 1-e 0+e],c3);plot([0 1 1 0 0],[0 0 1 1 0]);disp('weights');
  "IW{2,1}(35,:)'" : Constant  Value=[1.37495083195024481170776198268868029117584228515625;0.5483951907569404315978545128018595278263092041015625;-0.92242281176051010849192834939458407461643218994140625;-1.3360293949488666331859576530405320227146148681640625;1.409203748460716720813934443867765367031097412109375;0.532195298953798356933475588448345661163330078125;0.994814201859527624804968581884168088436126708984375;0.57804710526740932241551718107075430452823638916015625;0.05779605493124571891083718355730525217950344085693359375;-0.94377589100703407343218032110598869621753692626953125]
      mask Display: e = 0.06;c1 = [120 150 230]/255;c2 = ([120 150 230]+0)/383;c3 = ([120 150 230]+128)/383;patch([0 1 1 0],[0 0 1 1],c1);patch([0 1 1 1-e 1-e 0+e],[0 0 1 1-e 0+e 0+e],c2);patch([0 0 1 1-e 0+e 0+e],[0 1 1 1-e 1-e 0+e],c3);plot([0 1 1 0 0],[0 0 1 1 0]);disp('weights');
  "IW{2,1}(36,:)'" : Constant  Value=[1.269460142421657611322416414623148739337921142578125;-0.33101924650467251520780109785846434533596038818359375;-0.153329462238661395900862771668471395969390869140625;-1.1258490441263806491889454264310188591480255126953125;0.95503726339453376414923013726365752518177032470703125;-0.53555481618260036835721393799758516252040863037109375;-0.4550384158456612926357820470002479851245880126953125;1.1367000070454278404241676980745978653430938720703125;0.66211909557259363001691099270828999578952789306640625;1.8755139194223640064507208080613054335117340087890625]
      mask Display: e = 0.06;c1 = [120 150 230]/255;c2 = ([120 150 230]+0)/383;c3 = ([120 150 230]+128)/383;patch([0 1 1 0],[0 0 1 1],c1);patch([0 1 1 1-e 1-e 0+e],[0 0 1 1-e 0+e 0+e],c2);patch([0 0 1 1-e 0+e 0+e],[0 1 1 1-e 1-e 0+e],c3);plot([0 1 1 0 0],[0 0 1 1 0]);disp('weights');
  "IW{2,1}(37,:)'" : Constant  Value=[0.67899689065634716289565631086588837206363677978515625;0.497670322343243098917042743778438307344913482666015625;-1.3867411125638178237551301208441145718097686767578125;1.1512787975108025317894089312176220118999481201171875;0.0952459524952042613232805479128728620707988739013671875;-1.5565517945102509411725577592733316123485565185546875;0.27466587836181732829032853260287083685398101806640625;-0.32559826350659293314748765624244697391986846923828125;1.6513287904972802078162885663914494216442108154296875;-0.11269718547286032561682844743700115941464900970458984375]
      mask Display: e = 0.06;c1 = [120 150 230]/255;c2 = ([120 150 230]+0)/383;c3 = ([120 150 230]+128)/383;patch([0 1 1 0],[0 0 1 1],c1);patch([0 1 1 1-e 1-e 0+e],[0 0 1 1-e 0+e 0+e],c2);patch([0 0 1 1-e 0+e 0+e],[0 1 1 1-e 1-e 0+e],c3);plot([0 1 1 0 0],[0 0 1 1 0]);disp('weights');
  "IW{2,1}(38,:)'" : Constant  Value=[0.58007380698617883041379172937013208866119384765625;-0.37747275059312423994839491570019163191318511962890625;-1.2404015149491864899999882254633121192455291748046875;0.6682795874737179619984317469061352312564849853515625;0.704752316201355366587222306407056748867034912109375;-1.0695167638051075176264248511870391666889190673828125;0.1746369126049546471879381215330795384943485260009765625;1.197084545750607187386549412622116506099700927734375;1.39667954702562102653473630198277533054351806640625;1.6422663923751941172923807243932969868183135986328125]
      mask Display: e = 0.06;c1 = [120 150 230]/255;c2 = ([120 150 230]+0)/383;c3 = ([120 150 230]+128)/383;patch([0 1 1 0],[0 0 1 1],c1);patch([0 1 1 1-e 1-e 0+e],[0 0 1 1-e 0+e 0+e],c2);patch([0 0 1 1-e 0+e 0+e],[0 1 1 1-e 1-e 0+e],c3);plot([0 1 1 0 0],[0 0 1 1 0]);disp('weights');
  "IW{2,1}(39,:)'" : Constant  Value=[-0.393584510931811848433170553107629530131816864013671875;2.037226442566604678319208687753416597843170166015625;0.431093042992815866920608414147864095866680145263671875;-0.203097494395409416956255199693259783089160919189453125;1.7866530528206825412240732475765980780124664306640625;-1.9664522520547513817490425935829989612102508544921875;0.1692211099008324726167273865939932875335216522216796875;0.2741034365555343743636740327929146587848663330078125;0.5844218945474322080002593793324194848537445068359375;0.0003741402864169407482819451615796424448490142822265625]
      mask Display: e = 0.06;c1 = [120 150 230]/255;c2 = ([120 150 230]+0)/383;c3 = ([120 150 230]+128)/383;patch([0 1 1 0],[0 0 1 1],c1);patch([0 1 1 1-e 1-e 0+e],[0 0 1 1-e 0+e 0+e],c2);patch([0 0 1 1-e 0+e 0+e],[0 1 1 1-e 1-e 0+e],c3);plot([0 1 1 0 0],[0 0 1 1 0]);disp('weights');
  "IW{2,1}(4,:)'" : Constant  Value=[0.39535804463558921195698303563403896987438201904296875;0.6726256302466249170635137488716281950473785400390625;-0.379394796030003311759770667777047492563724517822265625;0.54703602924561101072953306356794200837612152099609375;1.722015158565024961490053101442754268646240234375;-0.59685980027987373119913172558881342411041259765625;2.5441008772744027055523474700748920440673828125;-0.016790141561619946475314435474501806311309337615966796875;1.1859700134984034747276382404379546642303466796875;-1.346403898530655229848207454779185354709625244140625]
      mask Display: e = 0.06;c1 = [120 150 230]/255;c2 = ([120 150 230]+0)/383;c3 = ([120 150 230]+128)/383;patch([0 1 1 0],[0 0 1 1],c1);patch([0 1 1 1-e 1-e 0+e],[0 0 1 1-e 0+e 0+e],c2);patch([0 0 1 1-e 0+e 0+e],[0 1 1 1-e 1-e 0+e],c3);plot([0 1 1 0 0],[0 0 1 1 0]);disp('weights');
  "IW{2,1}(40,:)'" : Constant  Value=[0.70094913082630860845512188461725600063800811767578125;1.6237173478412165739115380347357131540775299072265625;0.1613767235665594379501186494962894357740879058837890625;1.2413776837920325046837888294248841702938079833984375;0.90077145456603047168897546725929714739322662353515625;0.62131548616746190560888862819410860538482666015625;0.472202175411317204289929350125021301209926605224609375;0.40287344905192734589860492633306421339511871337890625;2.20162967136509823973256061435677111148834228515625;0.5000797645096570764877697001793421804904937744140625]
      mask Display: e = 0.06;c1 = [120 150 230]/255;c2 = ([120 150 230]+0)/383;c3 = ([120 150 230]+128)/383;patch([0 1 1 0],[0 0 1 1],c1);patch([0 1 1 1-e 1-e 0+e],[0 0 1 1-e 0+e 0+e],c2);patch([0 0 1 1-e 0+e 0+e],[0 1 1 1-e 1-e 0+e],c3);plot([0 1 1 0 0],[0 0 1 1 0]);disp('weights');
  "IW{2,1}(41,:)'" : Constant  Value=[0.89511272975841194021739966046879999339580535888671875;1.5390793265228468467142874942510388791561126708984375;-0.8356698244528164565281258546747267246246337890625;0.305111139376835815983923794192378409206867218017578125;1.618209786883517242728203200385905802249908447265625;-1.841739776980986231791348473052494227886199951171875;0.27122751900054631324366027911310084164142608642578125;-0.020576477298993811615446247742511332035064697265625;-0.34099555133854886346256307660951279103755950927734375;-0.491498629517409135747385562353883869946002960205078125]
      mask Display: e = 0.06;c1 = [120 150 230]/255;c2 = ([120 150 230]+0)/383;c3 = ([120 150 230]+128)/383;patch([0 1 1 0],[0 0 1 1],c1);patch([0 1 1 1-e 1-e 0+e],[0 0 1 1-e 0+e 0+e],c2);patch([0 0 1 1-e 0+e 0+e],[0 1 1 1-e 1-e 0+e],c3);plot([0 1 1 0 0],[0 0 1 1 0]);disp('weights');
  "IW{2,1}(42,:)'" : Constant  Value=[-0.408597028249068461303039612175780348479747772216796875;-0.2683588135376988592639690978103317320346832275390625;-0.1322439201414749021523675764910876750946044921875;-0.4786361148779498808636390094761736690998077392578125;0.0954746098104604368206338449454051442444324493408203125;-1.70734880160932878112589605734683573246002197265625;1.9989923181371473948075845328276045620441436767578125;-0.01348724535335532603852470856509171426296234130859375;1.2976940767067188797767585128895007073879241943359375;0.248389827143760955063811479703872464597225189208984375]
      mask Display: e = 0.06;c1 = [120 150 230]/255;c2 = ([120 150 230]+0)/383;c3 = ([120 150 230]+128)/383;patch([0 1 1 0],[0 0 1 1],c1);patch([0 1 1 1-e 1-e 0+e],[0 0 1 1-e 0+e 0+e],c2);patch([0 0 1 1-e 0+e 0+e],[0 1 1 1-e 1-e 0+e],c3);plot([0 1 1 0 0],[0 0 1 1 0]);disp('weights');
  "IW{2,1}(43,:)'" : Constant  Value=[0.112611486593226561847558286899584345519542694091796875;0.121761322384266235108185583158046938478946685791015625;-1.4633042066736814401650690342648886144161224365234375;-0.355278384048840101261390600484446622431278228759765625;-0.20455407079299536832195371971465647220611572265625;-2.0427413890000440943595094722695648670196533203125;1.0307631482155112934151475201360881328582763671875;-0.0974833344013328606525448094544117338955402374267578125;-0.2342737675588310863883378942773560993373394012451171875;0.78256760356682042445441993550048209726810455322265625]
      mask Display: e = 0.06;c1 = [120 150 230]/255;c2 = ([120 150 230]+0)/383;c3 = ([120 150 230]+128)/383;patch([0 1 1 0],[0 0 1 1],c1);patch([0 1 1 1-e 1-e 0+e],[0 0 1 1-e 0+e 0+e],c2);patch([0 0 1 1-e 0+e 0+e],[0 1 1 1-e 1-e 0+e],c3);plot([0 1 1 0 0],[0 0 1 1 0]);disp('weights');
  "IW{2,1}(44,:)'" : Constant  Value=[0.881902766611668997853712426149286329746246337890625;-0.251215810385145899008563219467760063707828521728515625;-1.2014645371899888015576607358525507152080535888671875;-0.770273748750251119332688176655210554599761962890625;-0.704433726648068248010758907184936106204986572265625;-1.1368347398115563606779687688685953617095947265625;1.022328284451336610771932100760750472545623779296875;0.64233488721398479537327830257709138095378875732421875;0.09024773019315457389666335075162351131439208984375;-0.03701232613250139691363216343233943916857242584228515625]
      mask Display: e = 0.06;c1 = [120 150 230]/255;c2 = ([120 150 230]+0)/383;c3 = ([120 150 230]+128)/383;patch([0 1 1 0],[0 0 1 1],c1);patch([0 1 1 1-e 1-e 0+e],[0 0 1 1-e 0+e 0+e],c2);patch([0 0 1 1-e 0+e 0+e],[0 1 1 1-e 1-e 0+e],c3);plot([0 1 1 0 0],[0 0 1 1 0]);disp('weights');
  "IW{2,1}(45,:)'" : Constant  Value=[-0.37139146307036530192391410309937782585620880126953125;0.29192364419080185644617131401901133358478546142578125;-1.418753126500496453132882379577495157718658447265625;-1.185858447948664462501255911774933338165283203125;0.1186785107654907689411771798404515720903873443603515625;-1.70793699167393153715011067106388509273529052734375;-0.1770807507842794559227428408121340908110141754150390625;-0.1241943409827283850699330969291622750461101531982421875;1.028402167385899179663510949467308819293975830078125;-0.1171737350662177268301178401088691316545009613037109375]
      mask Display: e = 0.06;c1 = [120 150 230]/255;c2 = ([120 150 230]+0)/383;c3 = ([120 150 230]+128)/383;patch([0 1 1 0],[0 0 1 1],c1);patch([0 1 1 1-e 1-e 0+e],[0 0 1 1-e 0+e 0+e],c2);patch([0 0 1 1-e 0+e 0+e],[0 1 1 1-e 1-e 0+e],c3);plot([0 1 1 0 0],[0 0 1 1 0]);disp('weights');
  "IW{2,1}(46,:)'" : Constant  Value=[1.036040256720980767823903079261071979999542236328125;1.15366598547695264898038658429868519306182861328125;-0.47739702059455979554769555761595256626605987548828125;-1.3371409868163548484432112672948278486728668212890625;0.4237074185437703643941631526104174554347991943359375;0.25388537756166240644262188652646727859973907470703125;0.63571474652533133120613229039008729159832000732421875;1.42838240164369256746113023837096989154815673828125;-0.012335098059212491750091800213340320624411106109619140625;-0.8216816360545333708387261140160262584686279296875]
      mask Display: e = 0.06;c1 = [120 150 230]/255;c2 = ([120 150 230]+0)/383;c3 = ([120 150 230]+128)/383;patch([0 1 1 0],[0 0 1 1],c1);patch([0 1 1 1-e 1-e 0+e],[0 0 1 1-e 0+e 0+e],c2);patch([0 0 1 1-e 0+e 0+e],[0 1 1 1-e 1-e 0+e],c3);plot([0 1 1 0 0],[0 0 1 1 0]);disp('weights');
  "IW{2,1}(47,:)'" : Constant  Value=[-0.6236764957015943355855824847822077572345733642578125;0.82270745091207542198930013910285197198390960693359375;-1.3885831767876977149711592574021779000759124755859375;-0.4152016460694059052372040241607464849948883056640625;0.8102624280102872500464172844658605754375457763671875;-0.6391319812874434180827165619120933115482330322265625;0.87511090616240794215485720997094176709651947021484375;1.573699281940742711327629876905120909214019775390625;-0.296018133536461558463770415983162820339202880859375;-0.49491811327092316563636131832026876509189605712890625]
      mask Display: e = 0.06;c1 = [120 150 230]/255;c2 = ([120 150 230]+0)/383;c3 = ([120 150 230]+128)/383;patch([0 1 1 0],[0 0 1 1],c1);patch([0 1 1 1-e 1-e 0+e],[0 0 1 1-e 0+e 0+e],c2);patch([0 0 1 1-e 0+e 0+e],[0 1 1 1-e 1-e 0+e],c3);plot([0 1 1 0 0],[0 0 1 1 0]);disp('weights');
  "IW{2,1}(48,:)'" : Constant  Value=[0.357332215682963194591792444043676368892192840576171875;1.253833758952895838234553593792952597141265869140625;0.6224463810640912253546730426023714244365692138671875;-1.0856176033105473521800377056933939456939697265625;0.2140251895549863669909740337971015833318233489990234375;-1.1253631570613100709721265957341529428958892822265625;1.4782574829530144011613401744398288428783416748046875;1.21925075602638788296872007776983082294464111328125;-0.228567268609606022433666794313467107713222503662109375;0.297512739048841512445875423509278334677219390869140625]
      mask Display: e = 0.06;c1 = [120 150 230]/255;c2 = ([120 150 230]+0)/383;c3 = ([120 150 230]+128)/383;patch([0 1 1 0],[0 0 1 1],c1);patch([0 1 1 1-e 1-e 0+e],[0 0 1 1-e 0+e 0+e],c2);patch([0 0 1 1-e 0+e 0+e],[0 1 1 1-e 1-e 0+e],c3);plot([0 1 1 0 0],[0 0 1 1 0]);disp('weights');
  "IW{2,1}(49,:)'" : Constant  Value=[0.75392413123939527874739496837719343602657318115234375;1.71805764610823619165103082195855677127838134765625;-0.42597619523504148819625925170839764177799224853515625;0.86870102444703489741328894524485804140567779541015625;-0.3357611476249662274540241924114525318145751953125;-1.4281404984240497757497223574318923056125640869140625;1.31708954914478226783103309571743011474609375;-0.1965562888633393956450134965052711777389049530029296875;1.8172017762036407617642908007837831974029541015625;0.399409637419585406004074457086971960961818695068359375]
      mask Display: e = 0.06;c1 = [120 150 230]/255;c2 = ([120 150 230]+0)/383;c3 = ([120 150 230]+128)/383;patch([0 1 1 0],[0 0 1 1],c1);patch([0 1 1 1-e 1-e 0+e],[0 0 1 1-e 0+e 0+e],c2);patch([0 0 1 1-e 0+e 0+e],[0 1 1 1-e 1-e 0+e],c3);plot([0 1 1 0 0],[0 0 1 1 0]);disp('weights');
  "IW{2,1}(5,:)'" : Constant  Value=[-0.8359417288208172980290555642568506300449371337890625;-0.485709998189083336228577536530792713165283203125;-2.076725329679750320366338200983591377735137939453125;-3.6054408917849283255918635404668748378753662109375;18.172813669848636664028163067996501922607421875;-14.7172963508549248246026763808913528919219970703125;5.5521758478126717051281957537867128849029541015625;11.123526129036651610704211634583771228790283203125;-3.257387883953123175473365336074493825435638427734375;-14.920565521218851046114650671370327472686767578125]
      mask Display: e = 0.06;c1 = [120 150 230]/255;c2 = ([120 150 230]+0)/383;c3 = ([120 150 230]+128)/383;patch([0 1 1 0],[0 0 1 1],c1);patch([0 1 1 1-e 1-e 0+e],[0 0 1 1-e 0+e 0+e],c2);patch([0 0 1 1-e 0+e 0+e],[0 1 1 1-e 1-e 0+e],c3);plot([0 1 1 0 0],[0 0 1 1 0]);disp('weights');
  "IW{2,1}(50,:)'" : Constant  Value=[0.285362623465485520934947771820588968694210052490234375;1.3178428096112517753368820194737054407596588134765625;0.417879419733507784240345017678919248282909393310546875;-0.585296256916358448307846629177220165729522705078125;-0.5577171531598745790603288696729578077793121337890625;-1.425666264391621584906033604056574404239654541015625;1.5587488217189557904163166313082911074161529541015625;0.79567837452157219590986869661719538271427154541015625;1.3987982597319723598872087677591480314731597900390625;0.8224235357057712025863338567432947456836700439453125]
      mask Display: e = 0.06;c1 = [120 150 230]/255;c2 = ([120 150 230]+0)/383;c3 = ([120 150 230]+128)/383;patch([0 1 1 0],[0 0 1 1],c1);patch([0 1 1 1-e 1-e 0+e],[0 0 1 1-e 0+e 0+e],c2);patch([0 0 1 1-e 0+e 0+e],[0 1 1 1-e 1-e 0+e],c3);plot([0 1 1 0 0],[0 0 1 1 0]);disp('weights');
  "IW{2,1}(51,:)'" : Constant  Value=[0.64066501778336171213368288590572774410247802734375;1.6663995182847834986006319013540633022785186767578125;0.47339537298517997410129964919178746640682220458984375;0.61336425689559093132885436716605909168720245361328125;0.64102663908356050104231371733476407825946807861328125;-0.259593402046055798937373992885113693773746490478515625;1.3194971171967193601659573687356896698474884033203125;0.34448692348508658245265223740716464817523956298828125;1.237207262515407801828359879436902701854705810546875;0.55136958662210844295259448699653148651123046875]
      mask Display: e = 0.06;c1 = [120 150 230]/255;c2 = ([120 150 230]+0)/383;c3 = ([120 150 230]+128)/383;patch([0 1 1 0],[0 0 1 1],c1);patch([0 1 1 1-e 1-e 0+e],[0 0 1 1-e 0+e 0+e],c2);patch([0 0 1 1-e 0+e 0+e],[0 1 1 1-e 1-e 0+e],c3);plot([0 1 1 0 0],[0 0 1 1 0]);disp('weights');
  "IW{2,1}(52,:)'" : Constant  Value=[0.0913045451772692973069212030168273486196994781494140625;0.72544031652523244257935175482998602092266082763671875;-0.221802982990443819932835367580992169678211212158203125;-1.35446651260686934392651892267167568206787109375;0.8379447782244564546516585323843173682689666748046875;-1.5918532639375022608163590120966546237468719482421875;-0.28343251609306630012241612348589114844799041748046875;-0.4322171809634769434893541983910836279392242431640625;1.49046350662874349524145145551301538944244384765625;-0.211801836229414452983377259442931972444057464599609375]
      mask Display: e = 0.06;c1 = [120 150 230]/255;c2 = ([120 150 230]+0)/383;c3 = ([120 150 230]+128)/383;patch([0 1 1 0],[0 0 1 1],c1);patch([0 1 1 1-e 1-e 0+e],[0 0 1 1-e 0+e 0+e],c2);patch([0 0 1 1-e 0+e 0+e],[0 1 1 1-e 1-e 0+e],c3);plot([0 1 1 0 0],[0 0 1 1 0]);disp('weights');
  "IW{2,1}(53,:)'" : Constant  Value=[-0.318464838094690672054554170244955457746982574462890625;-0.316918596347052716755143819682416506111621856689453125;-1.427882922259630760208892752416431903839111328125;0.72701404342009734449447933002375066280364990234375;2.4847218730205415937462021247483789920806884765625;-1.218668663666221618768759071826934814453125;-0.03802427933629330680798119601604412309825420379638671875;0.05559619116482784895172386541162268258631229400634765625;1.774446379456418032560804931563325226306915283203125;0.316617320318317851945977281502564437687397003173828125]
      mask Display: e = 0.06;c1 = [120 150 230]/255;c2 = ([120 150 230]+0)/383;c3 = ([120 150 230]+128)/383;patch([0 1 1 0],[0 0 1 1],c1);patch([0 1 1 1-e 1-e 0+e],[0 0 1 1-e 0+e 0+e],c2);patch([0 0 1 1-e 0+e 0+e],[0 1 1 1-e 1-e 0+e],c3);plot([0 1 1 0 0],[0 0 1 1 0]);disp('weights');
  "IW{2,1}(54,:)'" : Constant  Value=[1.4625583951700134033302447278401814401149749755859375;0.682890267125493277688974558259360492229461669921875;0.244312160599403138672158775079878978431224822998046875;0.289078167694109655627698884927667677402496337890625;-0.339985558240672336438592537888325750827789306640625;-0.450073136799514161854318672340014018118381500244140625;1.4971245329671629686885125920525752007961273193359375;-0.521119597906110509910604378092102706432342529296875;1.789740701333896399916056907386519014835357666015625;0.2661991865017807601390131821972317993640899658203125]
      mask Display: e = 0.06;c1 = [120 150 230]/255;c2 = ([120 150 230]+0)/383;c3 = ([120 150 230]+128)/383;patch([0 1 1 0],[0 0 1 1],c1);patch([0 1 1 1-e 1-e 0+e],[0 0 1 1-e 0+e 0+e],c2);patch([0 0 1 1-e 0+e 0+e],[0 1 1 1-e 1-e 0+e],c3);plot([0 1 1 0 0],[0 0 1 1 0]);disp('weights');
  "IW{2,1}(55,:)'" : Constant  Value=[0.910206005887114866226283993455581367015838623046875;-0.46559386637352873083983695323695428669452667236328125;-1.492358389852525224483770216465927660465240478515625;-1.73230265270798877708102736505679786205291748046875;1.4590505190877269825477924314327538013458251953125;-1.22137131656025932358033969649113714694976806640625;-0.3262557151888898498981461671064607799053192138671875;1.0585086356195276824365691936691291630268096923828125;-0.1069029675444712890186593767793965525925159454345703125;0.25951978925599206160512721908162347972393035888671875]
      mask Display: e = 0.06;c1 = [120 150 230]/255;c2 = ([120 150 230]+0)/383;c3 = ([120 150 230]+128)/383;patch([0 1 1 0],[0 0 1 1],c1);patch([0 1 1 1-e 1-e 0+e],[0 0 1 1-e 0+e 0+e],c2);patch([0 0 1 1-e 0+e 0+e],[0 1 1 1-e 1-e 0+e],c3);plot([0 1 1 0 0],[0 0 1 1 0]);disp('weights');
  "IW{2,1}(56,:)'" : Constant  Value=[0.44746845764097054054531099609448574483394622802734375;1.152696834936441039332066793576814234256744384765625;0.333685489259801515427028562044142745435237884521484375;-0.179288750532240415136442379662184976041316986083984375;0.95440760574506133817607178571051917970180511474609375;0.309199263350823427831670642262906767427921295166015625;0.31679280400718157206796377067803405225276947021484375;1.3126204015077698183944221455021761357784271240234375;1.463798375642620275272065555327571928501129150390625;1.64779603362415816292241288465447723865509033203125]
      mask Display: e = 0.06;c1 = [120 150 230]/255;c2 = ([120 150 230]+0)/383;c3 = ([120 150 230]+128)/383;patch([0 1 1 0],[0 0 1 1],c1);patch([0 1 1 1-e 1-e 0+e],[0 0 1 1-e 0+e 0+e],c2);patch([0 0 1 1-e 0+e 0+e],[0 1 1 1-e 1-e 0+e],c3);plot([0 1 1 0 0],[0 0 1 1 0]);disp('weights');
  "IW{2,1}(57,:)'" : Constant  Value=[0.7172315129687836243732590446597896516323089599609375;-0.457040040236674827145435529018868692219257354736328125;0.418517462705605247652584921524976380169391632080078125;-1.5388043006744538399033217501710169017314910888671875;1.6593402935871093273334508921834640204906463623046875;-0.1442640168449023929664321030941209755837917327880859375;0.52083034175381037744756440588389523327350616455078125;0.424966524365210485125743389289709739387035369873046875;1.436665904580655794831045568571425974369049072265625;1.12566044168118839507997108739800751209259033203125]
      mask Display: e = 0.06;c1 = [120 150 230]/255;c2 = ([120 150 230]+0)/383;c3 = ([120 150 230]+128)/383;patch([0 1 1 0],[0 0 1 1],c1);patch([0 1 1 1-e 1-e 0+e],[0 0 1 1-e 0+e 0+e],c2);patch([0 0 1 1-e 0+e 0+e],[0 1 1 1-e 1-e 0+e],c3);plot([0 1 1 0 0],[0 0 1 1 0]);disp('weights');
  "IW{2,1}(58,:)'" : Constant  Value=[0.81316480971366622565454918003524653613567352294921875;0.293717778141022289872807959909550845623016357421875;-1.4693292336168439771171279062400572001934051513671875;0.246310964947768551436269035548320971429347991943359375;0.70448897569881996361118581262417137622833251953125;-1.2954401474482539757815402481355704367160797119140625;1.2478146862325143473526622983627021312713623046875;-0.69747805719840105798112972479430027306079864501953125;-0.261026076045247246160130316638969816267490386962890625;0.9614659575549364678437314069014973938465118408203125]
      mask Display: e = 0.06;c1 = [120 150 230]/255;c2 = ([120 150 230]+0)/383;c3 = ([120 150 230]+128)/383;patch([0 1 1 0],[0 0 1 1],c1);patch([0 1 1 1-e 1-e 0+e],[0 0 1 1-e 0+e 0+e],c2);patch([0 0 1 1-e 0+e 0+e],[0 1 1 1-e 1-e 0+e],c3);plot([0 1 1 0 0],[0 0 1 1 0]);disp('weights');
  "IW{2,1}(59,:)'" : Constant  Value=[1.3901684878010651669200115065905265510082244873046875;0.74094955731323819403399966176948510110378265380859375;0.13063996819129852777763289850554428994655609130859375;-0.41548758734854140950432110912515781819820404052734375;1.7881989802444697712502374997711740434169769287109375;-0.8414261421537918561597280131536535918712615966796875;0.0737820833609433568422986127188778482377529144287109375;1.855516710898459376011260246741585433483123779296875;-0.1197290155807859968195572264448856003582477569580078125;-0.109854528976142507001867443250375799834728240966796875]
      mask Display: e = 0.06;c1 = [120 150 230]/255;c2 = ([120 150 230]+0)/383;c3 = ([120 150 230]+128)/383;patch([0 1 1 0],[0 0 1 1],c1);patch([0 1 1 1-e 1-e 0+e],[0 0 1 1-e 0+e 0+e],c2);patch([0 0 1 1-e 0+e 0+e],[0 1 1 1-e 1-e 0+e],c3);plot([0 1 1 0 0],[0 0 1 1 0]);disp('weights');
  "IW{2,1}(6,:)'" : Constant  Value=[1.5765510684902446225663652512594126164913177490234375;0.08210821512771275532127646101798745803534984588623046875;0.343625400134934533280528512477758340537548065185546875;-2.657253278266434204368806604179553687572479248046875;-0.019666581241213988706650894755512126721441745758056640625;0.53175686969345792309837861466803587973117828369140625;0.8325693862070266959563014097511768341064453125;1.6607623390166887933361294926726259291172027587890625;0.399917101709598987735461150805349461734294891357421875;-0.292198111503088220342050362887675873935222625732421875]
      mask Display: e = 0.06;c1 = [120 150 230]/255;c2 = ([120 150 230]+0)/383;c3 = ([120 150 230]+128)/383;patch([0 1 1 0],[0 0 1 1],c1);patch([0 1 1 1-e 1-e 0+e],[0 0 1 1-e 0+e 0+e],c2);patch([0 0 1 1-e 0+e 0+e],[0 1 1 1-e 1-e 0+e],c3);plot([0 1 1 0 0],[0 0 1 1 0]);disp('weights');
  "IW{2,1}(60,:)'" : Constant  Value=[0.2204500185427289704609421505665523000061511993408203125;0.42013793767149432145657783621572889387607574462890625;0.5673965149870685564792438526637852191925048828125;-0.04445656238629554224406348339471151120960712432861328125;0.69368994215888102328193554058088921010494232177734375;0.01364710502755454857304329152611899189651012420654296875;1.12774454930077894232454127632081508636474609375;1.2516526353363393031514760878053493797779083251953125;1.532365655078449240278359866351820528507232666015625;1.672399650123434167170444197836332023143768310546875]
      mask Display: e = 0.06;c1 = [120 150 230]/255;c2 = ([120 150 230]+0)/383;c3 = ([120 150 230]+128)/383;patch([0 1 1 0],[0 0 1 1],c1);patch([0 1 1 1-e 1-e 0+e],[0 0 1 1-e 0+e 0+e],c2);patch([0 0 1 1-e 0+e 0+e],[0 1 1 1-e 1-e 0+e],c3);plot([0 1 1 0 0],[0 0 1 1 0]);disp('weights');
  "IW{2,1}(61,:)'" : Constant  Value=[2.64938150173586262070557495462708175182342529296875;-2.631518895036423000277636674582026898860931396484375;-0.318246055292822960236520657417713664472103118896484375;-3.10227033638769711387794814072549343109130859375;2.00723967231829902857498382218182086944580078125;-2.8667569133943384684926058980636298656463623046875;3.090455093629757232776000819285400211811065673828125;2.003921052138760927618932328186929225921630859375;2.674742787378214803339915306423790752887725830078125;0.2239412155419397143507609371226863004267215728759765625]
      mask Display: e = 0.06;c1 = [120 150 230]/255;c2 = ([120 150 230]+0)/383;c3 = ([120 150 230]+128)/383;patch([0 1 1 0],[0 0 1 1],c1);patch([0 1 1 1-e 1-e 0+e],[0 0 1 1-e 0+e 0+e],c2);patch([0 0 1 1-e 0+e 0+e],[0 1 1 1-e 1-e 0+e],c3);plot([0 1 1 0 0],[0 0 1 1 0]);disp('weights');
  "IW{2,1}(62,:)'" : Constant  Value=[0.191624130396969183376398859763867221772670745849609375;0.2234925502306852884704113648695056326687335968017578125;-1.42292988856245816720047514536418020725250244140625;-1.6694138086123899711310514248907566070556640625;0.154120435025044077992362190343555994331836700439453125;0.2359710509488367191632818276048055849969387054443359375;0.828502814737149595458731710095889866352081298828125;-0.23409079351514383571242206016904674470424652099609375;1.2819919686532144087465212578536011278629302978515625;-0.8244365940854045948782413688604719936847686767578125]
      mask Display: e = 0.06;c1 = [120 150 230]/255;c2 = ([120 150 230]+0)/383;c3 = ([120 150 230]+128)/383;patch([0 1 1 0],[0 0 1 1],c1);patch([0 1 1 1-e 1-e 0+e],[0 0 1 1-e 0+e 0+e],c2);patch([0 0 1 1-e 0+e 0+e],[0 1 1 1-e 1-e 0+e],c3);plot([0 1 1 0 0],[0 0 1 1 0]);disp('weights');
  "IW{2,1}(63,:)'" : Constant  Value=[1.3399386681774050344984061666764318943023681640625;-0.11883600734961997924532539627762162126600742340087890625;0.4665247374149783521346535053453408181667327880859375;-2.445594414971620000898155922186560928821563720703125;1.363857088367332881517768328194506466388702392578125;0.2399630744271224191965785621505347080528736114501953125;0.403471789572983186022980817142524756491184234619140625;1.3883823012190623646944231950328685343265533447265625;0.32042540400551577928212054757750593125820159912109375;-0.1660133975818175733341064415071741677820682525634765625]
      mask Display: e = 0.06;c1 = [120 150 230]/255;c2 = ([120 150 230]+0)/383;c3 = ([120 150 230]+128)/383;patch([0 1 1 0],[0 0 1 1],c1);patch([0 1 1 1-e 1-e 0+e],[0 0 1 1-e 0+e 0+e],c2);patch([0 0 1 1-e 0+e 0+e],[0 1 1 1-e 1-e 0+e],c3);plot([0 1 1 0 0],[0 0 1 1 0]);disp('weights');
  "IW{2,1}(64,:)'" : Constant  Value=[0.6270756900528973165620527652208693325519561767578125;0.421626262659789030617929483923944644629955291748046875;-0.86382916272515064548542795819230377674102783203125;0.4868144993856897695394536640378646552562713623046875;2.30549250727704890806535331648774445056915283203125;-1.4107815131104983752408088548691011965274810791015625;-0.080552258424898715016837513758218847215175628662109375;0.93621745819690416201552807251573540270328521728515625;2.142748828105710767744085387676022946834564208984375;-0.451584105083504161459728720728890039026737213134765625]
      mask Display: e = 0.06;c1 = [120 150 230]/255;c2 = ([120 150 230]+0)/383;c3 = ([120 150 230]+128)/383;patch([0 1 1 0],[0 0 1 1],c1);patch([0 1 1 1-e 1-e 0+e],[0 0 1 1-e 0+e 0+e],c2);patch([0 0 1 1-e 0+e 0+e],[0 1 1 1-e 1-e 0+e],c3);plot([0 1 1 0 0],[0 0 1 1 0]);disp('weights');
  "IW{2,1}(65,:)'" : Constant  Value=[0.086180802669669154258969001602963544428348541259765625;-0.24446127642891202214059376274235546588897705078125;-1.45120770350726946418262741644866764545440673828125;0.021476378561471588801712329086512909270823001861572265625;0.5917675314292238919477995295892469584941864013671875;-1.6252456408582534042039924315758980810642242431640625;1.2074966170623075978340921210474334657192230224609375;0.9040277306821911107448386246687732636928558349609375;-0.44419863265848380518008298167842440307140350341796875;-0.11089192097159206173984102861140854656696319580078125]
      mask Display: e = 0.06;c1 = [120 150 230]/255;c2 = ([120 150 230]+0)/383;c3 = ([120 150 230]+128)/383;patch([0 1 1 0],[0 0 1 1],c1);patch([0 1 1 1-e 1-e 0+e],[0 0 1 1-e 0+e 0+e],c2);patch([0 0 1 1-e 0+e 0+e],[0 1 1 1-e 1-e 0+e],c3);plot([0 1 1 0 0],[0 0 1 1 0]);disp('weights');
  "IW{2,1}(66,:)'" : Constant  Value=[1.452275630180954291148509582853876054286956787109375;0.6159174155521836002691316025448031723499298095703125;-0.71262083567665968075743876397609710693359375;-1.051803807208672392192738698213361203670501708984375;1.250113974402875527403011801652610301971435546875;-1.133960028859494872932600628701038658618927001953125;-0.74788722144499708566200979475979693233966827392578125;0.7899568249485484638938714851974509656429290771484375;0.43498894790289688305762183517799712717533111572265625;0.349188606557321978840491283335722982883453369140625]
      mask Display: e = 0.06;c1 = [120 150 230]/255;c2 = ([120 150 230]+0)/383;c3 = ([120 150 230]+128)/383;patch([0 1 1 0],[0 0 1 1],c1);patch([0 1 1 1-e 1-e 0+e],[0 0 1 1-e 0+e 0+e],c2);patch([0 0 1 1-e 0+e 0+e],[0 1 1 1-e 1-e 0+e],c3);plot([0 1 1 0 0],[0 0 1 1 0]);disp('weights');
  "IW{2,1}(67,:)'" : Constant  Value=[1.306242746590990488897432442172430455684661865234375;0.55634185448419393171803903896943666040897369384765625;0.1195837798007045316150964708867832086980342864990234375;-1.9355192930022460107153392527834512293338775634765625;2.09472126903023170285678133950568735599517822265625;-0.70496675565883692993196518727927468717098236083984375;-0.257568888780242921665575295264716260135173797607421875;-0.1285102928746965911255273340429994277656078338623046875;0.74804718523463853419031011071638204157352447509765625;-0.328863363583867085448986244955449365079402923583984375]
      mask Display: e = 0.06;c1 = [120 150 230]/255;c2 = ([120 150 230]+0)/383;c3 = ([120 150 230]+128)/383;patch([0 1 1 0],[0 0 1 1],c1);patch([0 1 1 1-e 1-e 0+e],[0 0 1 1-e 0+e 0+e],c2);patch([0 0 1 1-e 0+e 0+e],[0 1 1 1-e 1-e 0+e],c3);plot([0 1 1 0 0],[0 0 1 1 0]);disp('weights');
  "IW{2,1}(68,:)'" : Constant  Value=[0.494614222684731263957047531221178360283374786376953125;0.47653421258267802951280600609607063233852386474609375;-0.2304139791360089450922288278889027424156665802001953125;-0.31583495965143659756080296574509702622890472412109375;1.963511086694238461092254510731436312198638916015625;-1.3564817962324162703424690334941260516643524169921875;-0.29631616190835219359911434366949833929538726806640625;1.7812857398150130361358378650038503110408782958984375;0.0950112565798066077693562192507670260965824127197265625;1.0286335224845435387663883375353179872035980224609375]
      mask Display: e = 0.06;c1 = [120 150 230]/255;c2 = ([120 150 230]+0)/383;c3 = ([120 150 230]+128)/383;patch([0 1 1 0],[0 0 1 1],c1);patch([0 1 1 1-e 1-e 0+e],[0 0 1 1-e 0+e 0+e],c2);patch([0 0 1 1-e 0+e 0+e],[0 1 1 1-e 1-e 0+e],c3);plot([0 1 1 0 0],[0 0 1 1 0]);disp('weights');
  "IW{2,1}(69,:)'" : Constant  Value=[1.515944879411889711917638123850338160991668701171875;-0.4351332482946344004659522397560067474842071533203125;-1.1767036778855588519121511126286350190639495849609375;0.342314712146432997830203248668112792074680328369140625;0.536093145523368175275891189812682569026947021484375;-0.97044400182899470674868780406541191041469573974609375;0.4325658625735628870501159326522611081600189208984375;1.46710108244449077830040550907142460346221923828125;0.349807104844269189936056818623910658061504364013671875;0.5586819363545088013012218652875162661075592041015625]
      mask Display: e = 0.06;c1 = [120 150 230]/255;c2 = ([120 150 230]+0)/383;c3 = ([120 150 230]+128)/383;patch([0 1 1 0],[0 0 1 1],c1);patch([0 1 1 1-e 1-e 0+e],[0 0 1 1-e 0+e 0+e],c2);patch([0 0 1 1-e 0+e 0+e],[0 1 1 1-e 1-e 0+e],c3);plot([0 1 1 0 0],[0 0 1 1 0]);disp('weights');
  "IW{2,1}(7,:)'" : Constant  Value=[-0.31815493343196166176056749463896267116069793701171875;-0.7689270346762546726182563361362554132938385009765625;-0.94144234988579100775751840046723373234272003173828125;-1.783774886522904612462525619775988161563873291015625;2.9931570206896385144546002265997231006622314453125;-1.640886537659195898442021643859334290027618408203125;0.89035738596309588199773088490474037826061248779296875;0.61176892691876372243342530055087991058826446533203125;-0.98233372810139607533841399344964884221553802490234375;-1.16841492782656519722195298527367413043975830078125]
      mask Display: e = 0.06;c1 = [120 150 230]/255;c2 = ([120 150 230]+0)/383;c3 = ([120 150 230]+128)/383;patch([0 1 1 0],[0 0 1 1],c1);patch([0 1 1 1-e 1-e 0+e],[0 0 1 1-e 0+e 0+e],c2);patch([0 0 1 1-e 0+e 0+e],[0 1 1 1-e 1-e 0+e],c3);plot([0 1 1 0 0],[0 0 1 1 0]);disp('weights');
  "IW{2,1}(70,:)'" : Constant  Value=[-0.61225848552345507602723273521405644714832305908203125;0.2350103297254114431691363051868393085896968841552734375;-0.7742110178931635999788340996019542217254638671875;1.145362298870285844287764120963402092456817626953125;2.048257236024020766507192092831246554851531982421875;-0.81795000736357703630119431181810796260833740234375;1.181119073224007554046011136961169540882110595703125;-0.316757588901413089654823806995409540832042694091796875;1.6976370131384062034385351580567657947540283203125;0.6308036418750606610927889050799421966075897216796875]
      mask Display: e = 0.06;c1 = [120 150 230]/255;c2 = ([120 150 230]+0)/383;c3 = ([120 150 230]+128)/383;patch([0 1 1 0],[0 0 1 1],c1);patch([0 1 1 1-e 1-e 0+e],[0 0 1 1-e 0+e 0+e],c2);patch([0 0 1 1-e 0+e 0+e],[0 1 1 1-e 1-e 0+e],c3);plot([0 1 1 0 0],[0 0 1 1 0]);disp('weights');
  "IW{2,1}(71,:)'" : Constant  Value=[0.204462636727950120008046042130445130169391632080078125;-0.2284366207356670341876991869867197237908840179443359375;-0.89295109061343092005103017072542570531368255615234375;0.135636740147973833270356180946691893041133880615234375;0.2451759214629051497613687615739763714373111724853515625;-1.1965294709892899671643817782751284539699554443359375;1.5298185230212248963965748771443031728267669677734375;1.223069543633053424258605446084402501583099365234375;-0.50314987147733447603314971274812705814838409423828125;1.415692961849842834709534145076759159564971923828125]
      mask Display: e = 0.06;c1 = [120 150 230]/255;c2 = ([120 150 230]+0)/383;c3 = ([120 150 230]+128)/383;patch([0 1 1 0],[0 0 1 1],c1);patch([0 1 1 1-e 1-e 0+e],[0 0 1 1-e 0+e 0+e],c2);patch([0 0 1 1-e 0+e 0+e],[0 1 1 1-e 1-e 0+e],c3);plot([0 1 1 0 0],[0 0 1 1 0]);disp('weights');
  "IW{2,1}(72,:)'" : Constant  Value=[0.40451033311711259710108379294979386031627655029296875;-0.195313512680955370104385337981511838734149932861328125;0.43806569883223012151773900768603198230266571044921875;0.060857786258460506989553806533876922912895679473876953125;0.5725443642207401762078688989276997745037078857421875;-0.8261145364308475347314697501133196055889129638671875;1.1405536549206072294282421353273093700408935546875;2.252623745411115319114969679503701627254486083984375;0.665747993629377532442958909086883068084716796875;0.14852630297200730691287162699154578149318695068359375]
      mask Display: e = 0.06;c1 = [120 150 230]/255;c2 = ([120 150 230]+0)/383;c3 = ([120 150 230]+128)/383;patch([0 1 1 0],[0 0 1 1],c1);patch([0 1 1 1-e 1-e 0+e],[0 0 1 1-e 0+e 0+e],c2);patch([0 0 1 1-e 0+e 0+e],[0 1 1 1-e 1-e 0+e],c3);plot([0 1 1 0 0],[0 0 1 1 0]);disp('weights');
  "IW{2,1}(73,:)'" : Constant  Value=[1.595209562017184889981535889091901481151580810546875;-0.64753260113876098813534554210491478443145751953125;-1.25408853822767696328810416162014007568359375;-0.5585706649786292832260414797929115593433380126953125;1.66442423476514012037341672112233936786651611328125;-2.56608626415569407441807925351895391941070556640625;0.65052673169134023201110039735794998705387115478515625;0.1623963713825300747561897196646896190941333770751953125;2.127271349496531183120850982959382236003875732421875;0.9288583423774372516135144906002096831798553466796875]
      mask Display: e = 0.06;c1 = [120 150 230]/255;c2 = ([120 150 230]+0)/383;c3 = ([120 150 230]+128)/383;patch([0 1 1 0],[0 0 1 1],c1);patch([0 1 1 1-e 1-e 0+e],[0 0 1 1-e 0+e 0+e],c2);patch([0 0 1 1-e 0+e 0+e],[0 1 1 1-e 1-e 0+e],c3);plot([0 1 1 0 0],[0 0 1 1 0]);disp('weights');
  "IW{2,1}(74,:)'" : Constant  Value=[-0.622638138934540119606708685751073062419891357421875;-1.0853918971993372633022545414860360324382781982421875;1.001712121416593159750618724501691758632659912109375;-0.07539729151186384814575802693070727400481700897216796875;-1.25258915923594127406204279395751655101776123046875;-0.2296387700225074046667117499964660964906215667724609375;-1.28269559918086439864737258176319301128387451171875;-0.63491579705198664118626084018615074455738067626953125;-0.398189490981556704074506569668301381170749664306640625;0.94401253610069935096049675848917104303836822509765625]
      mask Display: e = 0.06;c1 = [120 150 230]/255;c2 = ([120 150 230]+0)/383;c3 = ([120 150 230]+128)/383;patch([0 1 1 0],[0 0 1 1],c1);patch([0 1 1 1-e 1-e 0+e],[0 0 1 1-e 0+e 0+e],c2);patch([0 0 1 1-e 0+e 0+e],[0 1 1 1-e 1-e 0+e],c3);plot([0 1 1 0 0],[0 0 1 1 0]);disp('weights');
  "IW{2,1}(75,:)'" : Constant  Value=[-6.3001525218321461352388723753392696380615234375;-7.94817862774956207516652284539304673671722412109375;2.884437953447202662715653787017799913883209228515625;-13.4526352196139757921855562017299234867095947265625;-6.971098851473239932374781346879899501800537109375;6.319619383353636266065223026089370250701904296875;-6.0652264734902789911075160489417612552642822265625;-3.2158897180115300074021433829329907894134521484375;-6.943019068939438653842444182373583316802978515625;0.0720147632992167718857245972685632295906543731689453125]
      mask Display: e = 0.06;c1 = [120 150 230]/255;c2 = ([120 150 230]+0)/383;c3 = ([120 150 230]+128)/383;patch([0 1 1 0],[0 0 1 1],c1);patch([0 1 1 1-e 1-e 0+e],[0 0 1 1-e 0+e 0+e],c2);patch([0 0 1 1-e 0+e 0+e],[0 1 1 1-e 1-e 0+e],c3);plot([0 1 1 0 0],[0 0 1 1 0]);disp('weights');
  "IW{2,1}(76,:)'" : Constant  Value=[-0.251720994535631792388130634208209812641143798828125;-1.194258241738241022034117122530005872249603271484375;1.42516340105234373680787030025385320186614990234375;0.300872609336116869638289017530041746795177459716796875;-2.05024111137493303402834499138407409191131591796875;-0.1306887894187370446896778730661026202142238616943359375;0.005753569087534771142600220628082752227783203125;-0.91824383391391506403778066669474355876445770263671875;-0.183337548841915387587420127601944841444492340087890625;-0.96244018807980447061112272422178648412227630615234375]
      mask Display: e = 0.06;c1 = [120 150 230]/255;c2 = ([120 150 230]+0)/383;c3 = ([120 150 230]+128)/383;patch([0 1 1 0],[0 0 1 1],c1);patch([0 1 1 1-e 1-e 0+e],[0 0 1 1-e 0+e 0+e],c2);patch([0 0 1 1-e 0+e 0+e],[0 1 1 1-e 1-e 0+e],c3);plot([0 1 1 0 0],[0 0 1 1 0]);disp('weights');
  "IW{2,1}(77,:)'" : Constant  Value=[0.3778060004049812459214763293857686221599578857421875;-0.36885745543410963787067657904117368161678314208984375;-0.1372473167823594908387718760423013009130954742431640625;-0.8496248776603836372345313066034577786922454833984375;-1.7719740958063925351240186500945128500461578369140625;1.7033780946665857403132804392953403294086456298828125;-1.3984229944309209958674955487367697060108184814453125;-0.382308899524963774485541989633929915726184844970703125;-1.163670830261418043249932452454231679439544677734375;-1.0519319277071843554693941769073717296123504638671875]
      mask Display: e = 0.06;c1 = [120 150 230]/255;c2 = ([120 150 230]+0)/383;c3 = ([120 150 230]+128)/383;patch([0 1 1 0],[0 0 1 1],c1);patch([0 1 1 1-e 1-e 0+e],[0 0 1 1-e 0+e 0+e],c2);patch([0 0 1 1-e 0+e 0+e],[0 1 1 1-e 1-e 0+e],c3);plot([0 1 1 0 0],[0 0 1 1 0]);disp('weights');
  "IW{2,1}(78,:)'" : Constant  Value=[-1.12385152790150044666006579063832759857177734375;-0.7744663296753200310007514417520724236965179443359375;0.873628319266396946574104731553234159946441650390625;1.5156926812338678001168545961263589560985565185546875;-1.0212453100272345096755088889040052890777587890625;1.080628789462876770954835592419840395450592041015625;-0.232855606098379686041965896947658620774745941162109375;0.63743757833351188946124921130831353366374969482421875;-0.0567702784387111858421803844976238906383514404296875;0.0042332736038683538293270203212159685790538787841796875]
      mask Display: e = 0.06;c1 = [120 150 230]/255;c2 = ([120 150 230]+0)/383;c3 = ([120 150 230]+128)/383;patch([0 1 1 0],[0 0 1 1],c1);patch([0 1 1 1-e 1-e 0+e],[0 0 1 1-e 0+e 0+e],c2);patch([0 0 1 1-e 0+e 0+e],[0 1 1 1-e 1-e 0+e],c3);plot([0 1 1 0 0],[0 0 1 1 0]);disp('weights');
  "IW{2,1}(79,:)'" : Constant  Value=[-1.89560493895054360535823434474878013134002685546875;0.41210300107969566330012867183540947735309600830078125;0.0473552681309963030553689122825744561851024627685546875;0.721078680386060710816309438087046146392822265625;-1.87333798198959389225137783796526491641998291015625;1.79948011890404746537797109340317547321319580078125;-1.1129951828578885653087127138860523700714111328125;0.16371010132214591781263379743904806673526763916015625;-0.09690672730996287287386081743534305132925510406494140625;1.573727187671168703531066057621501386165618896484375]
      mask Display: e = 0.06;c1 = [120 150 230]/255;c2 = ([120 150 230]+0)/383;c3 = ([120 150 230]+128)/383;patch([0 1 1 0],[0 0 1 1],c1);patch([0 1 1 1-e 1-e 0+e],[0 0 1 1-e 0+e 0+e],c2);patch([0 0 1 1-e 0+e 0+e],[0 1 1 1-e 1-e 0+e],c3);plot([0 1 1 0 0],[0 0 1 1 0]);disp('weights');
  "IW{2,1}(8,:)'" : Constant  Value=[-0.5709479871845732912305493300664238631725311279296875;0.8536849040099478980181402221205644309520721435546875;-1.2479810829775157543508612434379756450653076171875;-0.71160329711020542386989973238087259232997894287109375;2.3785155115344966958446093485690653324127197265625;-0.91986637491216061146559468397754244506359100341796875;-0.00843559145879550775770638892936403863131999969482421875;0.406106567616938196607634381507523357868194580078125;0.78283436540703410511099491486675105988979339599609375;0.2230791823888085556593097180666518397629261016845703125]
      mask Display: e = 0.06;c1 = [120 150 230]/255;c2 = ([120 150 230]+0)/383;c3 = ([120 150 230]+128)/383;patch([0 1 1 0],[0 0 1 1],c1);patch([0 1 1 1-e 1-e 0+e],[0 0 1 1-e 0+e 0+e],c2);patch([0 0 1 1-e 0+e 0+e],[0 1 1 1-e 1-e 0+e],c3);plot([0 1 1 0 0],[0 0 1 1 0]);disp('weights');
  "IW{2,1}(80,:)'" : Constant  Value=[-1.1422280926079455554145170026458799839019775390625;0.706443133429740743878255671006627380847930908203125;1.049158523755867378213224583305418491363525390625;1.521244066087074298110337622347287833690643310546875;-1.6989197619802371974628840689547359943389892578125;1.0194007908390558814204496229649521410465240478515625;-0.87534004372401319482577264352585189044475555419921875;-0.60089932526064782081220982945524156093597412109375;0.45723949177882527994398742521298117935657501220703125;1.1717263085437235048402726533822715282440185546875]
      mask Display: e = 0.06;c1 = [120 150 230]/255;c2 = ([120 150 230]+0)/383;c3 = ([120 150 230]+128)/383;patch([0 1 1 0],[0 0 1 1],c1);patch([0 1 1 1-e 1-e 0+e],[0 0 1 1-e 0+e 0+e],c2);patch([0 0 1 1-e 0+e 0+e],[0 1 1 1-e 1-e 0+e],c3);plot([0 1 1 0 0],[0 0 1 1 0]);disp('weights');
  "IW{2,1}(81,:)'" : Constant  Value=[-1.555397195476971194949555865605361759662628173828125;0.1465059646955003958002095032497891224920749664306640625;1.290877223523276828842654140316881239414215087890625;-2.01740171287812142253415004233829677104949951171875;-1.908608307269882065071442411863245069980621337890625;1.436886324598578124067671524244360625743865966796875;-1.62167575976142952498548766016028821468353271484375;0.061822950587790137522148370408103801310062408447265625;-0.028982875339155278471281462771003134548664093017578125;0.12103140633771973522225806618735077790915966033935546875]
      mask Display: e = 0.06;c1 = [120 150 230]/255;c2 = ([120 150 230]+0)/383;c3 = ([120 150 230]+128)/383;patch([0 1 1 0],[0 0 1 1],c1);patch([0 1 1 1-e 1-e 0+e],[0 0 1 1-e 0+e 0+e],c2);patch([0 0 1 1-e 0+e 0+e],[0 1 1 1-e 1-e 0+e],c3);plot([0 1 1 0 0],[0 0 1 1 0]);disp('weights');
  "IW{2,1}(82,:)'" : Constant  Value=[-1.5274596916959997106033597447094507515430450439453125;-1.99158917846558569664239257690496742725372314453125;0.5793722601433923813374349265359342098236083984375;-0.5199954129321067153313151720794849097728729248046875;-0.528620645523072862914659708621911704540252685546875;1.146558714805799628067006779019720852375030517578125;-1.7329924979754711689139412555960007011890411376953125;0.220042104868850063592589094696450047194957733154296875;-0.1563284931892694462618464967817999422550201416015625;-0.193663433069747592529807889150106348097324371337890625]
      mask Display: e = 0.06;c1 = [120 150 230]/255;c2 = ([120 150 230]+0)/383;c3 = ([120 150 230]+128)/383;patch([0 1 1 0],[0 0 1 1],c1);patch([0 1 1 1-e 1-e 0+e],[0 0 1 1-e 0+e 0+e],c2);patch([0 0 1 1-e 0+e 0+e],[0 1 1 1-e 1-e 0+e],c3);plot([0 1 1 0 0],[0 0 1 1 0]);disp('weights');
  "IW{2,1}(83,:)'" : Constant  Value=[-1.8006623338624014873943224301910959184169769287109375;-0.00311237482679882493386003261548466980457305908203125;-0.36395138984239683299648504544165916740894317626953125;2.16204049450851965019637646037153899669647216796875;0.620935708677806008637389822979457676410675048828125;1.2372482385900787082988472320721484720706939697265625;-1.267031892992321218116558156907558441162109375;-0.88345798315537693579102551666437648236751556396484375;0.436077844842770456779135201941244304180145263671875;-0.22698178692355430730032139763352461159229278564453125]
      mask Display: e = 0.06;c1 = [120 150 230]/255;c2 = ([120 150 230]+0)/383;c3 = ([120 150 230]+128)/383;patch([0 1 1 0],[0 0 1 1],c1);patch([0 1 1 1-e 1-e 0+e],[0 0 1 1-e 0+e 0+e],c2);patch([0 0 1 1-e 0+e 0+e],[0 1 1 1-e 1-e 0+e],c3);plot([0 1 1 0 0],[0 0 1 1 0]);disp('weights');
  "IW{2,1}(84,:)'" : Constant  Value=[-0.85641615891905875646017420876887626945972442626953125;0.498595639617472941029774347043712623417377471923828125;1.4778936404946685367889358531101606786251068115234375;-0.5212632658390787820934519913862459361553192138671875;-0.9121117847776789577807221576222218573093414306640625;1.300533408939485102706612451584078371524810791015625;-0.4716553807738768089308223352418281137943267822265625;-0.3567424357827386760533272536122240126132965087890625;-1.4685566006438113273446788298315368592739105224609375;0.8754143981193671653073806737666018307209014892578125]
      mask Display: e = 0.06;c1 = [120 150 230]/255;c2 = ([120 150 230]+0)/383;c3 = ([120 150 230]+128)/383;patch([0 1 1 0],[0 0 1 1],c1);patch([0 1 1 1-e 1-e 0+e],[0 0 1 1-e 0+e 0+e],c2);patch([0 0 1 1-e 0+e 0+e],[0 1 1 1-e 1-e 0+e],c3);plot([0 1 1 0 0],[0 0 1 1 0]);disp('weights');
  "IW{2,1}(85,:)'" : Constant  Value=[-0.681223214996278247923555682064034044742584228515625;0.7478611420955509903052416120772249996662139892578125;-0.54570781212794428061130247442633844912052154541015625;1.158109130005175568811637276667170226573944091796875;-1.3021186757327052330168726257397793233394622802734375;1.602387014500834983010690848459489643573760986328125;-1.2091333171550455727327744170906953513622283935546875;0.277274414473033747885466482330230064690113067626953125;-0.9439897572231961131450361790484748780727386474609375;-1.2367602260799916980005264122155494987964630126953125]
      mask Display: e = 0.06;c1 = [120 150 230]/255;c2 = ([120 150 230]+0)/383;c3 = ([120 150 230]+128)/383;patch([0 1 1 0],[0 0 1 1],c1);patch([0 1 1 1-e 1-e 0+e],[0 0 1 1-e 0+e 0+e],c2);patch([0 0 1 1-e 0+e 0+e],[0 1 1 1-e 1-e 0+e],c3);plot([0 1 1 0 0],[0 0 1 1 0]);disp('weights');
  "IW{2,1}(86,:)'" : Constant  Value=[0.459045095515022649745873195570311509072780609130859375;-1.60416704811189614332533892593346536159515380859375;0.5405377596793827787990949218510650098323822021484375;-0.71078818957807554657080117976875044405460357666015625;1.146371418308608891578614930040203034877777099609375;1.012793186023221547742423354065977036952972412109375;-0.45302525365643919741387435351498425006866455078125;-0.62680731947356072009114313914324156939983367919921875;-1.9872778300235596216083422405063174664974212646484375;-0.82823941239589371487994640119723044335842132568359375]
      mask Display: e = 0.06;c1 = [120 150 230]/255;c2 = ([120 150 230]+0)/383;c3 = ([120 150 230]+128)/383;patch([0 1 1 0],[0 0 1 1],c1);patch([0 1 1 1-e 1-e 0+e],[0 0 1 1-e 0+e 0+e],c2);patch([0 0 1 1-e 0+e 0+e],[0 1 1 1-e 1-e 0+e],c3);plot([0 1 1 0 0],[0 0 1 1 0]);disp('weights');
  "IW{2,1}(87,:)'" : Constant  Value=[-0.235446160938551418695396932889707386493682861328125;-1.206580504799350084255138426669873297214508056640625;-0.80596304372118676706548967558774165809154510498046875;1.03114860350222681262266632984392344951629638671875;0.14698144965541926065810685031465254724025726318359375;1.0683540744214485851415474826353602111339569091796875;-0.6312008806060880328203666067565791308879852294921875;-0.426414186568314146352776106141391210258007049560546875;-1.610792750883007773410326990415342152118682861328125;0.1266141802539703931085313115545432083308696746826171875]
      mask Display: e = 0.06;c1 = [120 150 230]/255;c2 = ([120 150 230]+0)/383;c3 = ([120 150 230]+128)/383;patch([0 1 1 0],[0 0 1 1],c1);patch([0 1 1 1-e 1-e 0+e],[0 0 1 1-e 0+e 0+e],c2);patch([0 0 1 1-e 0+e 0+e],[0 1 1 1-e 1-e 0+e],c3);plot([0 1 1 0 0],[0 0 1 1 0]);disp('weights');
  "IW{2,1}(88,:)'" : Constant  Value=[0.53177489028717417340885731391608715057373046875;-0.0891257187073653811548723524538218043744564056396484375;-0.06301872435943135786207136561642982997000217437744140625;0.741559400299549142943078550160862505435943603515625;-1.6356022062199009337035704447771422564983367919921875;0.2194270220378019831120042226757504977285861968994140625;-0.3117911509623023658122065171482972800731658935546875;-0.431505321819778353553687111343606375157833099365234375;-2.196909816313290519929068977944552898406982421875;-1.27434260181343983475699133123271167278289794921875]
      mask Display: e = 0.06;c1 = [120 150 230]/255;c2 = ([120 150 230]+0)/383;c3 = ([120 150 230]+128)/383;patch([0 1 1 0],[0 0 1 1],c1);patch([0 1 1 1-e 1-e 0+e],[0 0 1 1-e 0+e 0+e],c2);patch([0 0 1 1-e 0+e 0+e],[0 1 1 1-e 1-e 0+e],c3);plot([0 1 1 0 0],[0 0 1 1 0]);disp('weights');
  "IW{2,1}(89,:)'" : Constant  Value=[-0.0813462808278463123112800303715630434453487396240234375;-0.510747728995242677996202473877929151058197021484375;0.75649368603254762977172731552855111658573150634765625;0.50137949238872547841339155638706870377063751220703125;-1.8536878017308058286261029934394173324108123779296875;0.496734125312879248870245874059037305414676666259765625;-0.78590924458719302325704347822465933859348297119140625;-1.03631763743176552594604800106026232242584228515625;-1.2043609655688547466212412473396398127079010009765625;-1.8831095326126703337621393075096420943737030029296875]
      mask Display: e = 0.06;c1 = [120 150 230]/255;c2 = ([120 150 230]+0)/383;c3 = ([120 150 230]+128)/383;patch([0 1 1 0],[0 0 1 1],c1);patch([0 1 1 1-e 1-e 0+e],[0 0 1 1-e 0+e 0+e],c2);patch([0 0 1 1-e 0+e 0+e],[0 1 1 1-e 1-e 0+e],c3);plot([0 1 1 0 0],[0 0 1 1 0]);disp('weights');
  "IW{2,1}(9,:)'" : Constant  Value=[1.5200486968993016656526151564321480691432952880859375;1.4662074784424639073421303692157380282878875732421875;-0.76705903337067049552189246242051012814044952392578125;1.6450601463993235196170417111716233193874359130859375;0.6252323345860071324153750538243912160396575927734375;-1.388264275396962954545188040356151759624481201171875;0.8835387754779218116851779996068216860294342041015625;-0.50735560835010129476785323276999406516551971435546875;0.364653673300981306937273984658531844615936279296875;2.391958634556393459291712133563123643398284912109375]
      mask Display: e = 0.06;c1 = [120 150 230]/255;c2 = ([120 150 230]+0)/383;c3 = ([120 150 230]+128)/383;patch([0 1 1 0],[0 0 1 1],c1);patch([0 1 1 1-e 1-e 0+e],[0 0 1 1-e 0+e 0+e],c2);patch([0 0 1 1-e 0+e 0+e],[0 1 1 1-e 1-e 0+e],c3);plot([0 1 1 0 0],[0 0 1 1 0]);disp('weights');
  "IW{2,1}(90,:)'" : Constant  Value=[-0.2117828993085375532956504684989340603351593017578125;-1.259226089325995445733497035689651966094970703125;1.2392355562773647026375556379207409918308258056640625;-0.435236273163499165494982889867969788610935211181640625;0.9174647615503668252046054476522840559482574462890625;0.9834960367290539462459264541394077241420745849609375;-0.001316065941896780999709193338276236318051815032958984375;-1.112413705800658902944633155129849910736083984375;-0.6404307699321034608175295943510718643665313720703125;-1.86081473541928321679961300105787813663482666015625]
      mask Display: e = 0.06;c1 = [120 150 230]/255;c2 = ([120 150 230]+0)/383;c3 = ([120 150 230]+128)/383;patch([0 1 1 0],[0 0 1 1],c1);patch([0 1 1 1-e 1-e 0+e],[0 0 1 1-e 0+e 0+e],c2);patch([0 0 1 1-e 0+e 0+e],[0 1 1 1-e 1-e 0+e],c3);plot([0 1 1 0 0],[0 0 1 1 0]);disp('weights');
  "IW{2,1}(91,:)'" : Constant  Value=[-2.70245616664291699038358274265192449092864990234375;-1.4588614675820499311242883777595125138759613037109375;0.7514928936934222036825303803198039531707763671875;-1.7521772353529030397112364880740642547607421875;-1.706978171034648994464077986776828765869140625;0.60307996520139084406508800384472124278545379638671875;-0.61725031771161187332808140126871876418590545654296875;0.47317466616297709780525337919243611395359039306640625;-0.582013314138770443406656340812332928180694580078125;0.339266867180890996369413414868176914751529693603515625]
      mask Display: e = 0.06;c1 = [120 150 230]/255;c2 = ([120 150 230]+0)/383;c3 = ([120 150 230]+128)/383;patch([0 1 1 0],[0 0 1 1],c1);patch([0 1 1 1-e 1-e 0+e],[0 0 1 1-e 0+e 0+e],c2);patch([0 0 1 1-e 0+e 0+e],[0 1 1 1-e 1-e 0+e],c3);plot([0 1 1 0 0],[0 0 1 1 0]);disp('weights');
  "IW{2,1}(92,:)'" : Constant  Value=[0.242587460385539188667536336652119643986225128173828125;0.325991692927507903387862597810453735291957855224609375;0.944027036437109945410384170827455818653106689453125;1.09583288134702794280883608735166490077972412109375;-1.424094148886367872108849041978828608989715576171875;-0.27066623168452863534838570558349601924419403076171875;-0.71172689482564843732603776516043581068515777587890625;-1.294788267032552564472780431970022618770599365234375;-0.32672464117209509826267321841442026197910308837890625;-1.6966469315208723145360636408440768718719482421875]
      mask Display: e = 0.06;c1 = [120 150 230]/255;c2 = ([120 150 230]+0)/383;c3 = ([120 150 230]+128)/383;patch([0 1 1 0],[0 0 1 1],c1);patch([0 1 1 1-e 1-e 0+e],[0 0 1 1-e 0+e 0+e],c2);patch([0 0 1 1-e 0+e 0+e],[0 1 1 1-e 1-e 0+e],c3);plot([0 1 1 0 0],[0 0 1 1 0]);disp('weights');
  "IW{2,1}(93,:)'" : Constant  Value=[-0.1891026330795331222844879448530264198780059814453125;1.1160757622300507829748994481633417308330535888671875;1.278695562440052668762291432358324527740478515625;-0.04338196706291040649627888114991947077214717864990234375;-0.1253924261545066032308426429153769277036190032958984375;0.8303294876258882073472022966598160564899444580078125;-1.114218102079637784385113263851962983608245849609375;-0.7951304332983168965398590444237925112247467041015625;-1.633340166452950104059027580660767853260040283203125;-1.24248360980409788822953487397171556949615478515625]
      mask Display: e = 0.06;c1 = [120 150 230]/255;c2 = ([120 150 230]+0)/383;c3 = ([120 150 230]+128)/383;patch([0 1 1 0],[0 0 1 1],c1);patch([0 1 1 1-e 1-e 0+e],[0 0 1 1-e 0+e 0+e],c2);patch([0 0 1 1-e 0+e 0+e],[0 1 1 1-e 1-e 0+e],c3);plot([0 1 1 0 0],[0 0 1 1 0]);disp('weights');
  "IW{2,1}(94,:)'" : Constant  Value=[-0.0287725593071444241122236462615546770393848419189453125;-2.25699404087468113999648267053999006748199462890625;-0.436908895089934856681423980262479744851589202880859375;-0.332432552921611612628538523495080880820751190185546875;0.85125201926890869952302409728872589766979217529296875;0.6481971198529705713298199043492786586284637451171875;-1.0443882428575019805094825642299838364124298095703125;-1.0909667550229189547650321401306428015232086181640625;-1.1136014763509722858003669898607768118381500244140625;-1.4555347128175133430971754933125339448451995849609375]
      mask Display: e = 0.06;c1 = [120 150 230]/255;c2 = ([120 150 230]+0)/383;c3 = ([120 150 230]+128)/383;patch([0 1 1 0],[0 0 1 1],c1);patch([0 1 1 1-e 1-e 0+e],[0 0 1 1-e 0+e 0+e],c2);patch([0 0 1 1-e 0+e 0+e],[0 1 1 1-e 1-e 0+e],c3);plot([0 1 1 0 0],[0 0 1 1 0]);disp('weights');
  "IW{2,1}(95,:)'" : Constant  Value=[-0.34202849002859803118070658456417731940746307373046875;-0.0184500522135545297341963077997206710278987884521484375;0.243746360908412451617977012574556283652782440185546875;1.3530755071326716620916386091266758739948272705078125;-2.01914108015383231276018705102615058422088623046875;0.90678895559900862810565058680367656052112579345703125;-1.2944034231759633524205810317653231322765350341796875;0.3048425957670135577615155852981843054294586181640625;-0.73467031884794009588546259692520834505558013916015625;1.7346760997713557284072294351062737405300140380859375]
      mask Display: e = 0.06;c1 = [120 150 230]/255;c2 = ([120 150 230]+0)/383;c3 = ([120 150 230]+128)/383;patch([0 1 1 0],[0 0 1 1],c1);patch([0 1 1 1-e 1-e 0+e],[0 0 1 1-e 0+e 0+e],c2);patch([0 0 1 1-e 0+e 0+e],[0 1 1 1-e 1-e 0+e],c3);plot([0 1 1 0 0],[0 0 1 1 0]);disp('weights');
  "IW{2,1}(96,:)'" : Constant  Value=[-0.4185556200349738187327375271706841886043548583984375;0.29518612217634554450995665320078842341899871826171875;1.605017380014584826852797050378285348415374755859375;1.273494461702679103609625599347054958343505859375;-1.5975499877662298064961987620336003601551055908203125;0.04469189356082599318131798327158321626484394073486328125;0.344404678363656291395500375074334442615509033203125;-0.5584747664291367375000163519871421158313751220703125;-0.2975689682256004164884188867290504276752471923828125;-1.371361564425833901026408057077787816524505615234375]
      mask Display: e = 0.06;c1 = [120 150 230]/255;c2 = ([120 150 230]+0)/383;c3 = ([120 150 230]+128)/383;patch([0 1 1 0],[0 0 1 1],c1);patch([0 1 1 1-e 1-e 0+e],[0 0 1 1-e 0+e 0+e],c2);patch([0 0 1 1-e 0+e 0+e],[0 1 1 1-e 1-e 0+e],c3);plot([0 1 1 0 0],[0 0 1 1 0]);disp('weights');
  "IW{2,1}(97,:)'" : Constant  Value=[-1.7030123402841617075154090343858115375041961669921875;0.2413925727986755698228904520874493755400180816650390625;0.2622618078893459436784496574546210467815399169921875;-0.8217037716875299491192663481342606246471405029296875;-3.1649623917139120266028839978389441967010498046875;1.0422134266039402294978799545788206160068511962890625;-1.0896693137877504486965563046396709978580474853515625;0.934528173771624448562533871154300868511199951171875;-1.2664303831960934676459373804391361773014068603515625;0.815860388837075678480914575629867613315582275390625]
      mask Display: e = 0.06;c1 = [120 150 230]/255;c2 = ([120 150 230]+0)/383;c3 = ([120 150 230]+128)/383;patch([0 1 1 0],[0 0 1 1],c1);patch([0 1 1 1-e 1-e 0+e],[0 0 1 1-e 0+e 0+e],c2);patch([0 0 1 1-e 0+e 0+e],[0 1 1 1-e 1-e 0+e],c3);plot([0 1 1 0 0],[0 0 1 1 0]);disp('weights');
  "IW{2,1}(98,:)'" : Constant  Value=[0.334106381596035173497938330910983495414257049560546875;0.001062028049707286481151413681800477206707000732421875;0.99597409674451464756117502474808134138584136962890625;1.3652607414237978300519671392976306378841400146484375;-1.5756802048072671151857093718717806041240692138671875;1.789025522615071306375966742052696645259857177734375;-0.37990559459124229046977916368632577359676361083984375;-1.118258980637407251634840577025897800922393798828125;-0.115730857815926457821120720836916007101535797119140625;-0.378326042072720969411392388792592100799083709716796875]
      mask Display: e = 0.06;c1 = [120 150 230]/255;c2 = ([120 150 230]+0)/383;c3 = ([120 150 230]+128)/383;patch([0 1 1 0],[0 0 1 1],c1);patch([0 1 1 1-e 1-e 0+e],[0 0 1 1-e 0+e 0+e],c2);patch([0 0 1 1-e 0+e 0+e],[0 1 1 1-e 1-e 0+e],c3);plot([0 1 1 0 0],[0 0 1 1 0]);disp('weights');
  "IW{2,1}(99,:)'" : Constant  Value=[-2.1745880608445968817932225647382438182830810546875;-1.867791634890526797363463629153557121753692626953125;1.0911096493650280780940420299884863197803497314453125;-0.511988986458684625091564157628454267978668212890625;-2.9473037650332827297461335547268390655517578125;2.43908129976606158351160047459416091442108154296875;-0.68958251693137995186333455421845428645610809326171875;-1.350275371743186791917423761333338916301727294921875;0.041221249314860937407178909097638097591698169708251953125;-0.435559498738867956202369668972096405923366546630859375]
      mask Display: e = 0.06;c1 = [120 150 230]/255;c2 = ([120 150 230]+0)/383;c3 = ([120 150 230]+128)/383;patch([0 1 1 0],[0 0 1 1],c1);patch([0 1 1 1-e 1-e 0+e],[0 0 1 1-e 0+e 0+e],c2);patch([0 0 1 1-e 0+e 0+e],[0 1 1 1-e 1-e 0+e],c3);plot([0 1 1 0 0],[0 0 1 1 0]);disp('weights');
  Mux : Mux  Inputs=131
      mask Display: e = 0.06;c1 = [120 150 230]/255;c2 = ([120 150 230]+0)/383;c3 = ([120 150 230]+128)/383;patch([0 1 1 0],[0 0 1 1],c1);patch([0 1 1 1-e 1-e 0+e],[0 0 1 1-e 0+e 0+e],c2);patch([0 0 1 1-e 0+e 0+e],[0 1 1 1-e 1-e 0+e],c3);plot([0 1 1 0 0],[0 0 1 1 0]);disp('Mux');
  dotprod{1..131} (131 alike) : neural/Weight Functions/dotprod  SystemSampleTime=-1
  "lz{2,1}" : Outport
      mask Display: e = 0.06;c1 = [120 230 180]/255;c2 = ([120 230 180]+0)/(256+128);c3 = ([120 230 180]+128)/(256+128);patch([0 1 1 0],[0 0 1 1],c1);patch([0 1 1 1-e 1-e 0+e],[0 0 1 1-e 0+e 0+e],c2);patch([0 0 1 1-e 0+e 0+e],[0 1 1 1-e 1-e 0+e],c3);plot([0 1 1 0 0],[0 0 1 1 0]);
  wires:
  "IW{2,1}(1,:)'"/1 -> dotprod1/1
  "ad{2,1}"/1 -> dotprod1/2, dotprod2/2, dotprod3/2, dotprod4/2, dotprod5/2, dotprod6/2, dotprod7/2, dotprod8/2, dotprod9/2, dotprod10/2, dotprod11/2, dotprod12/2, dotprod13/2, dotprod14/2, dotprod15/2, dotprod16/2, dotprod17/2, dotprod18/2, dotprod19/2, dotprod20/2, dotprod21/2, dotprod22/2, dotprod23/2, dotprod24/2, dotprod25/2, dotprod26/2, dotprod27/2, dotprod28/2, dotprod29/2, dotprod30/2, dotprod31/2, dotprod32/2, dotprod33/2, dotprod34/2, dotprod35/2, dotprod36/2, dotprod37/2, dotprod38/2, dotprod39/2, dotprod40/2, dotprod41/2, dotprod42/2, dotprod43/2, dotprod44/2, dotprod45/2, dotprod46/2, dotprod47/2, dotprod48/2, dotprod49/2, dotprod50/2, dotprod51/2, dotprod52/2, dotprod53/2, dotprod54/2, dotprod55/2, dotprod56/2, dotprod57/2, dotprod58/2, dotprod59/2, dotprod60/2, dotprod61/2, dotprod62/2, dotprod63/2, dotprod64/2, dotprod65/2, dotprod66/2, dotprod67/2, dotprod68/2, dotprod69/2, dotprod70/2, dotprod71/2, dotprod72/2, dotprod73/2, dotprod74/2, dotprod75/2, dotprod76/2, dotprod77/2, dotprod78/2, dotprod79/2, dotprod80/2, dotprod81/2, dotprod82/2, dotprod83/2, dotprod84/2, dotprod85/2, dotprod86/2, dotprod87/2, dotprod88/2, dotprod89/2, dotprod90/2, dotprod91/2, dotprod92/2, dotprod93/2, dotprod94/2, dotprod95/2, dotprod96/2, dotprod97/2, dotprod98/2, dotprod99/2, dotprod100/2, dotprod101/2, dotprod102/2, dotprod103/2, dotprod104/2, dotprod105/2, dotprod106/2, dotprod107/2, dotprod108/2, dotprod109/2, dotprod110/2, dotprod111/2, dotprod112/2, dotprod113/2, dotprod114/2, dotprod115/2, dotprod116/2, dotprod117/2, dotprod118/2, dotprod119/2, dotprod120/2, dotprod121/2, dotprod122/2, dotprod123/2, dotprod124/2, dotprod125/2, dotprod126/2, dotprod127/2, dotprod128/2, dotprod129/2, dotprod130/2, dotprod131/2
  dotprod1/1 -> Mux/1
  "IW{2,1}(2,:)'"/1 -> dotprod2/1
  dotprod2/1 -> Mux/2
  "IW{2,1}(3,:)'"/1 -> dotprod3/1
  dotprod3/1 -> Mux/3
  "IW{2,1}(4,:)'"/1 -> dotprod4/1
  dotprod4/1 -> Mux/4
  "IW{2,1}(5,:)'"/1 -> dotprod5/1
  dotprod5/1 -> Mux/5
  "IW{2,1}(6,:)'"/1 -> dotprod6/1
  dotprod6/1 -> Mux/6
  "IW{2,1}(7,:)'"/1 -> dotprod7/1
  dotprod7/1 -> Mux/7
  "IW{2,1}(8,:)'"/1 -> dotprod8/1
  dotprod8/1 -> Mux/8
  "IW{2,1}(9,:)'"/1 -> dotprod9/1
  dotprod9/1 -> Mux/9
  "IW{2,1}(10,:)'"/1 -> dotprod10/1
  dotprod10/1 -> Mux/10
  "IW{2,1}(11,:)'"/1 -> dotprod11/1
  dotprod11/1 -> Mux/11
  "IW{2,1}(12,:)'"/1 -> dotprod12/1
  dotprod12/1 -> Mux/12
  "IW{2,1}(13,:)'"/1 -> dotprod13/1
  dotprod13/1 -> Mux/13
  "IW{2,1}(14,:)'"/1 -> dotprod14/1
  dotprod14/1 -> Mux/14
  "IW{2,1}(15,:)'"/1 -> dotprod15/1
  dotprod15/1 -> Mux/15
  "IW{2,1}(16,:)'"/1 -> dotprod16/1
  dotprod16/1 -> Mux/16
  "IW{2,1}(17,:)'"/1 -> dotprod17/1
  dotprod17/1 -> Mux/17
  "IW{2,1}(18,:)'"/1 -> dotprod18/1
  dotprod18/1 -> Mux/18
  "IW{2,1}(19,:)'"/1 -> dotprod19/1
  dotprod19/1 -> Mux/19
  "IW{2,1}(20,:)'"/1 -> dotprod20/1
  dotprod20/1 -> Mux/20
  "IW{2,1}(21,:)'"/1 -> dotprod21/1
  dotprod21/1 -> Mux/21
  "IW{2,1}(22,:)'"/1 -> dotprod22/1
  dotprod22/1 -> Mux/22
  "IW{2,1}(23,:)'"/1 -> dotprod23/1
  dotprod23/1 -> Mux/23
  "IW{2,1}(24,:)'"/1 -> dotprod24/1
  dotprod24/1 -> Mux/24
  "IW{2,1}(25,:)'"/1 -> dotprod25/1
  dotprod25/1 -> Mux/25
  "IW{2,1}(26,:)'"/1 -> dotprod26/1
  dotprod26/1 -> Mux/26
  "IW{2,1}(27,:)'"/1 -> dotprod27/1
  dotprod27/1 -> Mux/27
  "IW{2,1}(28,:)'"/1 -> dotprod28/1
  dotprod28/1 -> Mux/28
  "IW{2,1}(29,:)'"/1 -> dotprod29/1
  dotprod29/1 -> Mux/29
  "IW{2,1}(30,:)'"/1 -> dotprod30/1
  dotprod30/1 -> Mux/30
  "IW{2,1}(31,:)'"/1 -> dotprod31/1
  dotprod31/1 -> Mux/31
  "IW{2,1}(32,:)'"/1 -> dotprod32/1
  dotprod32/1 -> Mux/32
  "IW{2,1}(33,:)'"/1 -> dotprod33/1
  dotprod33/1 -> Mux/33
  "IW{2,1}(34,:)'"/1 -> dotprod34/1
  dotprod34/1 -> Mux/34
  "IW{2,1}(35,:)'"/1 -> dotprod35/1
  dotprod35/1 -> Mux/35
  "IW{2,1}(36,:)'"/1 -> dotprod36/1
  dotprod36/1 -> Mux/36
  "IW{2,1}(37,:)'"/1 -> dotprod37/1
  dotprod37/1 -> Mux/37
  "IW{2,1}(38,:)'"/1 -> dotprod38/1
  dotprod38/1 -> Mux/38
  "IW{2,1}(39,:)'"/1 -> dotprod39/1
  dotprod39/1 -> Mux/39
  "IW{2,1}(40,:)'"/1 -> dotprod40/1
  dotprod40/1 -> Mux/40
  "IW{2,1}(41,:)'"/1 -> dotprod41/1
  dotprod41/1 -> Mux/41
  "IW{2,1}(42,:)'"/1 -> dotprod42/1
  dotprod42/1 -> Mux/42
  "IW{2,1}(43,:)'"/1 -> dotprod43/1
  dotprod43/1 -> Mux/43
  "IW{2,1}(44,:)'"/1 -> dotprod44/1
  dotprod44/1 -> Mux/44
  "IW{2,1}(45,:)'"/1 -> dotprod45/1
  dotprod45/1 -> Mux/45
  "IW{2,1}(46,:)'"/1 -> dotprod46/1
  dotprod46/1 -> Mux/46
  "IW{2,1}(47,:)'"/1 -> dotprod47/1
  dotprod47/1 -> Mux/47
  "IW{2,1}(48,:)'"/1 -> dotprod48/1
  dotprod48/1 -> Mux/48
  "IW{2,1}(49,:)'"/1 -> dotprod49/1
  dotprod49/1 -> Mux/49
  "IW{2,1}(50,:)'"/1 -> dotprod50/1
  dotprod50/1 -> Mux/50
  "IW{2,1}(51,:)'"/1 -> dotprod51/1
  dotprod51/1 -> Mux/51
  "IW{2,1}(52,:)'"/1 -> dotprod52/1
  dotprod52/1 -> Mux/52
  "IW{2,1}(53,:)'"/1 -> dotprod53/1
  dotprod53/1 -> Mux/53
  "IW{2,1}(54,:)'"/1 -> dotprod54/1
  dotprod54/1 -> Mux/54
  "IW{2,1}(55,:)'"/1 -> dotprod55/1
  dotprod55/1 -> Mux/55
  "IW{2,1}(56,:)'"/1 -> dotprod56/1
  dotprod56/1 -> Mux/56
  "IW{2,1}(57,:)'"/1 -> dotprod57/1
  dotprod57/1 -> Mux/57
  "IW{2,1}(58,:)'"/1 -> dotprod58/1
  dotprod58/1 -> Mux/58
  "IW{2,1}(59,:)'"/1 -> dotprod59/1
  dotprod59/1 -> Mux/59
  "IW{2,1}(60,:)'"/1 -> dotprod60/1
  dotprod60/1 -> Mux/60
  "IW{2,1}(61,:)'"/1 -> dotprod61/1
  dotprod61/1 -> Mux/61
  "IW{2,1}(62,:)'"/1 -> dotprod62/1
  dotprod62/1 -> Mux/62
  "IW{2,1}(63,:)'"/1 -> dotprod63/1
  dotprod63/1 -> Mux/63
  "IW{2,1}(64,:)'"/1 -> dotprod64/1
  dotprod64/1 -> Mux/64
  "IW{2,1}(65,:)'"/1 -> dotprod65/1
  dotprod65/1 -> Mux/65
  "IW{2,1}(66,:)'"/1 -> dotprod66/1
  dotprod66/1 -> Mux/66
  "IW{2,1}(67,:)'"/1 -> dotprod67/1
  dotprod67/1 -> Mux/67
  "IW{2,1}(68,:)'"/1 -> dotprod68/1
  dotprod68/1 -> Mux/68
  "IW{2,1}(69,:)'"/1 -> dotprod69/1
  dotprod69/1 -> Mux/69
  "IW{2,1}(70,:)'"/1 -> dotprod70/1
  dotprod70/1 -> Mux/70
  "IW{2,1}(71,:)'"/1 -> dotprod71/1
  dotprod71/1 -> Mux/71
  "IW{2,1}(72,:)'"/1 -> dotprod72/1
  dotprod72/1 -> Mux/72
  "IW{2,1}(73,:)'"/1 -> dotprod73/1
  dotprod73/1 -> Mux/73
  "IW{2,1}(74,:)'"/1 -> dotprod74/1
  dotprod74/1 -> Mux/74
  "IW{2,1}(75,:)'"/1 -> dotprod75/1
  dotprod75/1 -> Mux/75
  "IW{2,1}(76,:)'"/1 -> dotprod76/1
  dotprod76/1 -> Mux/76
  "IW{2,1}(77,:)'"/1 -> dotprod77/1
  dotprod77/1 -> Mux/77
  "IW{2,1}(78,:)'"/1 -> dotprod78/1
  dotprod78/1 -> Mux/78
  "IW{2,1}(79,:)'"/1 -> dotprod79/1
  dotprod79/1 -> Mux/79
  "IW{2,1}(80,:)'"/1 -> dotprod80/1
  dotprod80/1 -> Mux/80
  "IW{2,1}(81,:)'"/1 -> dotprod81/1
  dotprod81/1 -> Mux/81
  "IW{2,1}(82,:)'"/1 -> dotprod82/1
  dotprod82/1 -> Mux/82
  "IW{2,1}(83,:)'"/1 -> dotprod83/1
  dotprod83/1 -> Mux/83
  "IW{2,1}(84,:)'"/1 -> dotprod84/1
  dotprod84/1 -> Mux/84
  "IW{2,1}(85,:)'"/1 -> dotprod85/1
  dotprod85/1 -> Mux/85
  "IW{2,1}(86,:)'"/1 -> dotprod86/1
  dotprod86/1 -> Mux/86
  "IW{2,1}(87,:)'"/1 -> dotprod87/1
  dotprod87/1 -> Mux/87
  "IW{2,1}(88,:)'"/1 -> dotprod88/1
  dotprod88/1 -> Mux/88
  "IW{2,1}(89,:)'"/1 -> dotprod89/1
  dotprod89/1 -> Mux/89
  "IW{2,1}(90,:)'"/1 -> dotprod90/1
  dotprod90/1 -> Mux/90
  "IW{2,1}(91,:)'"/1 -> dotprod91/1
  dotprod91/1 -> Mux/91
  "IW{2,1}(92,:)'"/1 -> dotprod92/1
  dotprod92/1 -> Mux/92
  "IW{2,1}(93,:)'"/1 -> dotprod93/1
  dotprod93/1 -> Mux/93
  "IW{2,1}(94,:)'"/1 -> dotprod94/1
  dotprod94/1 -> Mux/94
  "IW{2,1}(95,:)'"/1 -> dotprod95/1
  dotprod95/1 -> Mux/95
  "IW{2,1}(96,:)'"/1 -> dotprod96/1
  dotprod96/1 -> Mux/96
  "IW{2,1}(97,:)'"/1 -> dotprod97/1
  dotprod97/1 -> Mux/97
  "IW{2,1}(98,:)'"/1 -> dotprod98/1
  dotprod98/1 -> Mux/98
  "IW{2,1}(99,:)'"/1 -> dotprod99/1
  dotprod99/1 -> Mux/99
  "IW{2,1}(100,:)'"/1 -> dotprod100/1
  dotprod100/1 -> Mux/100
  "IW{2,1}(101,:)'"/1 -> dotprod101/1
  dotprod101/1 -> Mux/101
  "IW{2,1}(102,:)'"/1 -> dotprod102/1
  dotprod102/1 -> Mux/102
  "IW{2,1}(103,:)'"/1 -> dotprod103/1
  dotprod103/1 -> Mux/103
  "IW{2,1}(104,:)'"/1 -> dotprod104/1
  dotprod104/1 -> Mux/104
  "IW{2,1}(105,:)'"/1 -> dotprod105/1
  dotprod105/1 -> Mux/105
  "IW{2,1}(106,:)'"/1 -> dotprod106/1
  dotprod106/1 -> Mux/106
  "IW{2,1}(107,:)'"/1 -> dotprod107/1
  dotprod107/1 -> Mux/107
  "IW{2,1}(108,:)'"/1 -> dotprod108/1
  dotprod108/1 -> Mux/108
  "IW{2,1}(109,:)'"/1 -> dotprod109/1
  dotprod109/1 -> Mux/109
  "IW{2,1}(110,:)'"/1 -> dotprod110/1
  dotprod110/1 -> Mux/110
  "IW{2,1}(111,:)'"/1 -> dotprod111/1
  dotprod111/1 -> Mux/111
  "IW{2,1}(112,:)'"/1 -> dotprod112/1
  dotprod112/1 -> Mux/112
  "IW{2,1}(113,:)'"/1 -> dotprod113/1
  dotprod113/1 -> Mux/113
  "IW{2,1}(114,:)'"/1 -> dotprod114/1
  dotprod114/1 -> Mux/114
  "IW{2,1}(115,:)'"/1 -> dotprod115/1
  dotprod115/1 -> Mux/115
  "IW{2,1}(116,:)'"/1 -> dotprod116/1
  dotprod116/1 -> Mux/116
  "IW{2,1}(117,:)'"/1 -> dotprod117/1
  dotprod117/1 -> Mux/117
  "IW{2,1}(118,:)'"/1 -> dotprod118/1
  dotprod118/1 -> Mux/118
  "IW{2,1}(119,:)'"/1 -> dotprod119/1
  dotprod119/1 -> Mux/119
  "IW{2,1}(120,:)'"/1 -> dotprod120/1
  dotprod120/1 -> Mux/120
  "IW{2,1}(121,:)'"/1 -> dotprod121/1
  dotprod121/1 -> Mux/121
  "IW{2,1}(122,:)'"/1 -> dotprod122/1
  dotprod122/1 -> Mux/122
  "IW{2,1}(123,:)'"/1 -> dotprod123/1
  dotprod123/1 -> Mux/123
  "IW{2,1}(124,:)'"/1 -> dotprod124/1
  dotprod124/1 -> Mux/124
  "IW{2,1}(125,:)'"/1 -> dotprod125/1
  dotprod125/1 -> Mux/125
  "IW{2,1}(126,:)'"/1 -> dotprod126/1
  dotprod126/1 -> Mux/126
  "IW{2,1}(127,:)'"/1 -> dotprod127/1
  dotprod127/1 -> Mux/127
  "IW{2,1}(128,:)'"/1 -> dotprod128/1
  dotprod128/1 -> Mux/128
  "IW{2,1}(129,:)'"/1 -> dotprod129/1
  dotprod129/1 -> Mux/129
  "IW{2,1}(130,:)'"/1 -> dotprod130/1
  dotprod130/1 -> Mux/130
  "IW{2,1}(131,:)'"/1 -> dotprod131/1
  dotprod131/1 -> Mux/131
  Mux/1 -> "lz{2,1}"/1
